simulink library "pmm"  (R2021b)
settings: Solver=VariableStepAuto  StartTime=0.0  StopTime=10.0  RelTol=1e-3
undefined symbols (not defined in the file or in its folder): APMM_CoolgFanActCurr_X_pct, APMM_EWP1Curr_X_c, APMM_EWP3Curr_X_c, APMM_LVBattChktime_X_enum, APMM_LVBattChrgtime_X_enum, APMM_LVChrgLv24V_X_mV, APMM_LVChrgLv_X_mV, ENUM_ANTITHEFT_ALARM, ENUM_ANTITHEFT_ARM, ENUM_ANTITHEFT_DISARM, ENUM_ANTITHEFT_WAIT, ENUM_CHRGPLUGSTA_NONE, ENUM_CRASHSTATE_NOCRASH, ENUM_DCDCFAULTSTA_ANYFAULTLV1, ENUM_DCDCFAULTSTA_ANYFAULTLV2, ENUM_DRIVETRAIN_AWD, ENUM_DRIVETRAIN_FWD, ENUM_DRIVETRAIN_RWD, ENUM_EBSBRKSW_PRESSED, ENUM_GEARACTUALPOSN_D, ENUM_GEARACTUALPOSN_N, ENUM_GEARACTUALPOSN_P, ENUM_GEARACTUALPOSN_R, ENUM_HVBATTREADYPRE_READY, ENUM_PDKEYRAWLULOCK_INLOCK, ENUM_PDKEYRAWLULOCK_INUNLOCK, ENUM_PDKEYRAWPS_INPS, ENUM_PDKEYSTA_LOCK, ENUM_PDKEYSTA_PS, ENUM_PDKEYSTA_UNAVALIABLE, ENUM_PDKEYSTA_UNLOCK, ENUM_POWERSTA_OFF, ENUM_POWERSTA_OFFA, ENUM_POWERSTA_OFFC, ENUM_POWERSTA_ON, ENUM_POWERSTA_READY, ENUM_POWERSTA_STANDBY, ENUM_PWRSTASW_PWRUP, ENUM_PWRSTASW_READY, FALSE, KPMM_AllDoorClosedHoldTime_s, KPMM_APSAllowThd_pct, KPMM_BattDownFailtime_s, KPMM_BattUpFailtime_s, KPMM_BattUpResetRty_cnt, KPMM_BattUpResetSW_flg, KPMM_BattUpResetTO_s, KPMM_BattUpRstDlyTO_s, KPMM_BrakeSWHoldTime_s, KPMM_ChrgPlugHoldTime_s, KPMM_DCDCDisableFailtime_s, KPMM_DCDCEnableFailtime_s, KPMM_DCDCVSET_V, KPMM_DCDCVSETLVChrg_V, KPMM_DoorSWHoldTime_s, KPMM_DriverSafetyChkFailtime_s, KPMM_DrivetrainSelect_enum_ovrdflg, KPMM_DrivetrainSelect_enum_ovrdval, KPMM_FDADC12VDetAccu_s, KPMM_FDADC12VDetAccuIntval_s ... (+60)
libraries: simulink x35, hcu_lib x13
(part 5 of 6)

== stateflow chart pmm/PMM/PMM/PMM_State_Machine ==
  state OFF
    en:
    VPMM_LVPwrSta_flg = FALSE;
    VPMM_PowerSta_enum = ENUM_POWERSTA_OFF;
    VPMM_PwrStaSW_enum = ENUM_PWRSTASW_OFF;
    VPMM_LVSilentChrgSta_enum = ENUM_SILENTCHRGSTA_NONE;
    VPMM_LVSilentChrgReq_flg = FALSE;
    VPMM_LVSilentChrgReqStd_flg = FALSE;
    VPMM_PreOFF_flg = TRUE;
    VPMM_PwrStaTOSta_enum = ENUM_PWRSTATOSTA_NORMAL;
    VPMM_PowerUpState_enum = ENUM_PUSTATE_INITIALIZE;
    VPMM_FirstLVCheckHoldTimer_s = 0;
    VPMM_24VFirstLVCheckHoldTimer_s = 0;
    VPMM_PMMAllowECUSleep_flg = FALSE;
    VPMM_SilentChrgFaultBypass_flg = FALSE;
    VPMM_FDADC12VDetAvg_mV = 0;
    VPMM_FDADC24VDetAvg_mV = 0;
    VPMM_SilentChkAllowSleep_flg = FALSE;
    ex:
    VPMM_PMMAllowECUSleep_flg = FALSE;
    VPMM_PMMAllowNMSleep_flg = FALSE;
    state LVBatt_Check_Wake_Hold [parallel]
      en:
      VPMM_LVBattChkWakeholdTimer_s = 0;
      VPMM_TimerAllowSleep_flg = FALSE;
      settings: executionOrder=1
      (default) -> (junction 3132)
      (junction 3132) -> (junction 3133) [order 1] : [VPMM_LVBattChkWakeholdTimer_s >= KPMM_LVBattChkWakehold_s]
      LVBatt_Check_Wake_Hold -> (junction 3132)
      (junction 3132) -> (junction 3134) [order 2] : {
          |  VPMM_LVBattChkWakeholdTimer_s += task_time_s;
          |  VPMM_TimerAllowSleep_flg = FALSE;
          | }
      (junction 3133) -> (junction 3135) : {VPMM_TimerAllowSleep_flg = TRUE;
          |  VPMM_LVBattChkWakeholdTimer_s = KPMM_LVBattChkWakehold_s;}
      (junction 3135) -> (junction 3134)
    state Silent_Charge_Judge [parallel]
      en:
      VPMM_SilentChkAllowSleep12V_flg = FALSE;
      settings: executionOrder=2
      state SilentChrgLv = SilentChrgLvCal(LVBatt_mV) [function]
      state LVBatStaChk
        en:
        VPMM_FDADC12VDetAccuTimer_s = 0;
        VPMM_OFFLVBattChkRechk_cnt = 0;
        VPMM_FDADC12VDetAccu_cnt = 0;
        VPMM_FDADC12VDetbuff_mV = 0;
        VPMM_FDADC12VDetAvgTMP_mV = 0;
        VPMM_OFFLVBattChkRechkDone_flg = FALSE;
        VPMM_LVBatStaChk_flg = 0;
        (default) -> (junction 3179)
        OFF.Silent_Charge_Judge.LVBatStaChk -> (junction 3179) [order 1]
        (junction 3179) -> (junction 3180) [order 1] : [VPMM_FirstLVCheckHoldTimer_s >= KPMM_FirstLVCheckHoldT_s]
        (junction 3180) -> (junction 3181) : {VPMM_FirstLVCheckHoldTimer_s = KPMM_FirstLVCheckHoldT_s;}
        (junction 3179) -> (junction 3195) [order 2] : {
            |  VPMM_FirstLVCheckHoldTimer_s += task_time_s;
            |  VPMM_OFFLVBattChkRechkDone_flg = FALSE;
            |  VPMM_SilentChkAllowSleep12V_flg = FALSE;
            |  }
        (junction 3181) -> (junction 3182) [order 1] : [VPMM_FDADC12VDetAccuTimer_s >= ...
            | (VPMM_FDADC12VDetAccu_cnt * KPMM_FDADC12VDetAccuIntval_s)]
        (junction 3181) -> (junction 3183) [order 2]
        (junction 3182) -> (junction 3184) : {VPMM_FDADC12VDetbuff_mV += VINP_LvBattVolt_mV;
            |  VPMM_FDADC12VDetAccu_cnt++;}
        (junction 3184) -> (junction 3183)
        (junction 3183) -> (junction 3185)
        (junction 3185) -> (junction 3186) [order 1] : [VPMM_FDADC12VDetAccuTimer_s >= KPMM_FDADC12VDetAccu_s]
        (junction 3185) -> (junction 3196) [order 2] : {VPMM_FDADC12VDetAccuTimer_s += task_time_s;}
        (junction 3186) -> (junction 3405)
        (junction 3405) -> (junction 3406) [order 1] : [VPMM_FDADC12VDetAccu_cnt <= 0]
        (junction 3405) -> (junction 3410) [order 2] : {VPMM_FDADC12VDetAvgTMP_mV = VPMM_FDADC12VDetbuff_mV / VPMM_FDADC12VDetAccu_cnt;}
        (junction 3406) -> (junction 3412) : {VPMM_FDADC12VDetAvgTMP_mV = VINP_LvBattVolt_mV;}
        (junction 3412) -> (junction 3410)
        (junction 3410) -> (junction 3187)
        (junction 3187) -> (junction 3188) [order 1] : [VPMM_FirstFDADC12VDetAvg_mV <= 0]
        (junction 3187) -> (junction 3189) [order 2]
        (junction 3188) -> (junction 3190) : {VPMM_FirstFDADC12VDetAvg_mV = VPMM_FDADC12VDetAvgTMP_mV;}
        (junction 3190) -> (junction 3189)
        (junction 3189) -> (junction 3191) : {VPMM_FDADC12VDetAvg_mV = VPMM_FDADC12VDetAvgTMP_mV;}
        (junction 3191) -> (junction 3192) [order 1] : [VPMM_FDADC12VDetAvgTMP_mV < KPMM_LVBattOFFSlpThd_mV]
        (junction 3191) -> (junction 3197) [order 2] : {
            |  VPMM_LVBatStaChk_flg = TRUE;
            | }
        (junction 3192) -> (junction 3193) : {VPMM_LVBatStaChk_flg = FALSE;}
        (junction 3193) -> (junction 3194) [order 1] : [VPMM_OFFLVBattChkRechk_cnt >= KPMM_OFFLVBattChkRetry_cnt ]
        (junction 3193) -> (junction 3198) [order 2] : {
            |  VPMM_OFFLVBattChkRechkDone_flg = FALSE;
            |  VPMM_OFFLVBattChkRechk_cnt++;
            |  VPMM_FDADC12VDetAccuTimer_s = 0;
            |  VPMM_FDADC12VDetAccu_cnt = 0;
            |  VPMM_FDADC12VDetbuff_mV = 0;
            |  VPMM_FDADC12VDetAvgTMP_mV = 0;}
        (junction 3194) -> (junction 3199) : {VPMM_OFFLVBattChkRechkDone_flg = TRUE;}
        (junction 3196) -> (junction 3195)
        (junction 3197) -> (junction 3196)
        (junction 3198) -> (junction 3197)
        (junction 3199) -> (junction 3198)
      state HoodOffStaChk [commented out]
        en:
        VPMM_HoodOffStaChk_flg = FALSE;
        (default) -> (junction 3255) [commented out] : {VPMM_HoodOffChkFailtimer_s = 0;}
        OFF.Silent_Charge_Judge.HoodOffStaChk -> (junction 3255) [commented out]
        (junction 3255) -> (junction 3256) [commented out] : [!VINP_HoodSW_flg]
        (junction 3256) -> (junction 3258) [commented out] : {VPMM_HoodOffStaChk_flg = TRUE;}
        (junction 3255) -> (junction 3257) [commented out] : {VPMM_HoodOffChkFailtimer_s += task_time_s;}
        (junction 3258) -> (junction 3257) [commented out]
        (junction 3257) -> (junction 3259) [commented out]
      state CANMsgValid
        en:
        VPMM_CANMsgValid_flg = FALSE;
        (default) -> (junction 3229) : {VPMM_CANValidChkFailtimer_s = 0;}
        OFF.Silent_Charge_Judge.CANMsgValid -> (junction 3229) [order 1]
        (junction 3229) -> (junction 3230) [order 1] : [VINP_CANMsgValidBMS3_flg && VINP_CANMsgValidBMS5_flg]
        (junction 3229) -> (junction 3231) [order 2] : {VPMM_CANValidChkFailtimer_s += task_time_s;}
        (junction 3230) -> (junction 3232) : {VPMM_CANMsgValid_flg = TRUE;}
        (junction 3232) -> (junction 3231)
        (junction 3231) -> (junction 3233)
      state HVBSOCOffStaChk
        en:
        VPMM_HVBSOCOffStaChk_flg = FALSE;
        (default) -> (junction 3242) : {VPMM_HVBSOCOffStaChkFailtimer_s = 0;}
        (junction 3242) -> (junction 3243) [order 1] : [VINP_HVBattSOC_pct > KPMM_HVBattSOCThd_pct]
        OFF.Silent_Charge_Judge.HVBSOCOffStaChk -> (junction 3242) [order 1]
        (junction 3242) -> (junction 3244) [order 2] : {VPMM_HVBSOCOffStaChkFailtimer_s += task_time_s;}
        (junction 3243) -> (junction 3245) : {VPMM_HVBSOCOffStaChk_flg = TRUE;}
        (junction 3245) -> (junction 3244)
        (junction 3244) -> (junction 3246)
      state Silent_Charge_Allow_Sleep
        en:
        VPMM_LVSilentChrgLv12V_enum = SilentChrgLvCal(VPMM_FDADC12VDetAvg_mV);
        VPMM_SilentChkAllowSleep12V_flg = TRUE;
        VPMM_LVSilentChrgReq12V_flg = FALSE;
        VPMM_PMMAllowNMSleep12V_flg = TRUE;
      state Silent_Charge_Need_Wake
        en:
        VPMM_LVSilentChrgLv12V_enum = SilentChrgLvCal(VPMM_FDADC12VDetAvg_mV);
        %VPMM_LVChrgReqCnt_cnt++;
        VPMM_SilentChkAllowSleep12V_flg = FALSE;
        VPMM_LVSilentChrgReq12V_flg = TRUE;
      (default) -> (junction 3144)
      (junction 3143) -> (junction 3144)
      (junction 3144) -> (junction 3145) [order 1] : [!KPMM_OFFStaByPassLVBatt_flg]
      (junction 3150) -> (junction 3143)
      (junction 3144) -> OFF.Silent_Charge_Judge.Silent_Charge_Allow_Sleep [order 2]
      (junction 3145) -> OFF.Silent_Charge_Judge.LVBatStaChk
      OFF.Silent_Charge_Judge.LVBatStaChk -> (junction 3146) [order 2] : [VPMM_LVBatStaChk_flg == TRUE]
      (junction 3146) -> (junction 3149)
      OFF.Silent_Charge_Judge.LVBatStaChk -> (junction 3438) [order 1] : [VPMM_LVBatStaChk_flg == FALSE &&...
          |  VPMM_OFFLVBattChkRechkDone_flg == TRUE]
      (junction 3149) -> (junction 3440)
      OFF.Silent_Charge_Judge.HoodOffStaChk -> ? [commented out] : [VPMM_HoodOffChkFailtimer_s >= KPMM_HoodOffChkFailtime_s]
          | {VPMM_LVSilentChrgSta_enum = ENUM_SILENTCHRGSTA_FAULT;}
      OFF.Silent_Charge_Judge.HoodOffStaChk -> ? [commented out] : [VPMM_HoodOffStaChk_flg]
      (junction 3438) -> (junction 3440) [commented out] : [VPMM_SilentChrgFaultBypass_flg]
      (junction 3438) -> OFF.Silent_Charge_Judge.CANMsgValid : {VPMM_PMMAllowNMSleep12V_flg = FALSE;}
      (junction 3440) -> (junction 3147)
      OFF.Silent_Charge_Judge.CANMsgValid -> (junction 3147) [order 2] : [VPMM_CANValidChkFailtimer_s >= KPMM_CANValidChkFailtime_s]
          | {VPMM_LVSilentChrgSta_enum = ENUM_SILENTCHRGSTA_FAULT;
          |  VPMM_SilentChrgFaultBypass_flg = TRUE;}
      (junction 3147) -> (junction 3148)
      OFF.Silent_Charge_Judge.CANMsgValid -> OFF.Silent_Charge_Judge.HVBSOCOffStaChk [order 1] : [VPMM_CANMsgValid_flg]
      OFF.Silent_Charge_Judge.HVBSOCOffStaChk -> (junction 3148) [order 2] : [VPMM_HVBSOCOffStaChkFailtimer_s >= KPMM_HVBSOCOffStaChkFailtime_s]
          | {VPMM_LVSilentChrgSta_enum = ENUM_SILENTCHRGSTA_FAULT;
          |  VPMM_SilentChrgFaultBypass_flg = TRUE;}
      (junction 3148) -> (junction 3355)
      OFF.Silent_Charge_Judge.HVBSOCOffStaChk -> (junction 3354) [order 1] : [VPMM_HVBSOCOffStaChk_flg]
      (junction 3354) -> (junction 3355) [order 2] : {VPMM_LVSilentChrgSta_enum = ENUM_SILENTCHRGSTA_FAULT;
          |  VPMM_SilentChrgFaultBypass_flg = TRUE;}
      (junction 3355) -> OFF.Silent_Charge_Judge.Silent_Charge_Allow_Sleep
      (junction 3354) -> OFF.Silent_Charge_Judge.Silent_Charge_Need_Wake [order 1] : [VPMM_PowerUpFault_enum == ENUM_PUFAULT_NOFAULT]
      OFF.Silent_Charge_Judge.Silent_Charge_Allow_Sleep -> (junction 3151)
      OFF.Silent_Charge_Judge.Silent_Charge_Need_Wake -> (junction 3152)
      (junction 3151) -> (junction 3150)
      (junction 3152) -> (junction 3151)
    state Silent_Charge_Judge24V [parallel]
      en:
      VPMM_SilentChkAllowSleep24V_flg = FALSE;
      settings: executionOrder=3
      state SilentChrgLv24V = SilentChrgLvCal24V(LVBatt24V_mV) [function]
      state LVBatStaChk
        en:
        VPMM_FDADC24VDetAccuTimer_s = 0;
        VPMM_24VOFFLVBattChkRechk_cnt = 0;
        VPMM_FDADC24VDetAccu_cnt = 0;
        VPMM_FDADC24VDetbuff_mV = 0;
        VPMM_FDADC24VDetAvgTMP_mV = 0;
        VPMM_24VOFFLVBattChkRechkDone_flg = FALSE;
        VPMM_24VLVBatStaChk_flg = 0;
        (default) -> (junction 3872)
        OFF.Silent_Charge_Judge24V.LVBatStaChk -> (junction 3872) [order 1]
        (junction 3872) -> (junction 3873) [order 1] : [VPMM_24VFirstLVCheckHoldTimer_s >= KPMM_FirstLVCheckHoldT_s]
        (junction 3872) -> (junction 3892) [order 2] : {
            |  VPMM_24VFirstLVCheckHoldTimer_s += task_time_s;
            |  VPMM_24VOFFLVBattChkRechkDone_flg = FALSE;
            |  VPMM_SilentChkAllowSleep24V_flg = FALSE;
            |  }
        (junction 3873) -> (junction 3874) : {VPMM_24VFirstLVCheckHoldTimer_s = KPMM_FirstLVCheckHoldT_s;}
        (junction 3874) -> (junction 3875) [order 1] : [VPMM_FDADC24VDetAccuTimer_s >= ...
            | (VPMM_FDADC24VDetAccu_cnt * KPMM_FDADC24VDetAccuIntval_s)]
        (junction 3874) -> (junction 3876) [order 2]
        (junction 3875) -> (junction 3877) : {VPMM_FDADC24VDetbuff_mV += VINP_LvBattVolt24V_mV;
            |  VPMM_FDADC24VDetAccu_cnt++;}
        (junction 3877) -> (junction 3876)
        (junction 3876) -> (junction 3878)
        (junction 3878) -> (junction 3879) [order 1] : [VPMM_FDADC24VDetAccuTimer_s >= KPMM_FDADC24VDetAccu_s]
        (junction 3878) -> (junction 3893) [order 2] : {VPMM_FDADC24VDetAccuTimer_s += task_time_s;}
        (junction 3879) -> (junction 3880)
        (junction 3880) -> (junction 3881) [order 1] : [VPMM_FDADC24VDetAccu_cnt <= 0]
        (junction 3880) -> (junction 3882) [order 2] : {VPMM_FDADC24VDetAvgTMP_mV = VPMM_FDADC24VDetbuff_mV / VPMM_FDADC24VDetAccu_cnt;}
        (junction 3881) -> (junction 3883) : {VPMM_FDADC24VDetAvgTMP_mV = VINP_LvBattVolt24V_mV;}
        (junction 3883) -> (junction 3882)
        (junction 3882) -> (junction 3884)
        (junction 3884) -> (junction 3885) [order 1] : [VPMM_FirstFDADC24VDetAvg_mV <= 0]
        (junction 3884) -> (junction 3886) [order 2]
        (junction 3885) -> (junction 3887) : {VPMM_FirstFDADC24VDetAvg_mV = VPMM_FDADC24VDetAvgTMP_mV;}
        (junction 3887) -> (junction 3886)
        (junction 3886) -> (junction 3888) : {VPMM_FDADC24VDetAvg_mV = VPMM_FDADC24VDetAvgTMP_mV;}
        (junction 3888) -> (junction 3889) [order 1] : [VPMM_FDADC24VDetAvgTMP_mV < KPMM_LVBattOFFSlpThd24V_mV]
        (junction 3888) -> (junction 3894) [order 2] : {
            |  VPMM_24VLVBatStaChk_flg = TRUE;
            | }
        (junction 3889) -> (junction 3890) : {VPMM_24VLVBatStaChk_flg = FALSE;}
        (junction 3890) -> (junction 3891) [order 1] : [VPMM_24VOFFLVBattChkRechk_cnt >= KPMM_OFFLVBattChkRetry_cnt ]
        (junction 3890) -> (junction 3895) [order 2] : {
            |  VPMM_24VOFFLVBattChkRechkDone_flg = FALSE;
            |  VPMM_24VOFFLVBattChkRechk_cnt++;
            |  VPMM_FDADC24VDetAccuTimer_s = 0;
            |  VPMM_FDADC24VDetAccu_cnt = 0;
            |  VPMM_FDADC24VDetbuff_mV = 0;
            |  VPMM_FDADC24VDetAvgTMP_mV = 0;}
        (junction 3891) -> (junction 3896) : {VPMM_24VOFFLVBattChkRechkDone_flg = TRUE;}
        (junction 3893) -> (junction 3892)
        (junction 3894) -> (junction 3893)
        (junction 3895) -> (junction 3894)
        (junction 3896) -> (junction 3895)
      state HoodOffStaChk [commented out]
        en:
        VPMM_HoodOffStaChk_flg = FALSE;
        (default) -> (junction 3931) [commented out] : {VPMM_HoodOffChkFailtimer_s = 0;}
        OFF.Silent_Charge_Judge24V.HoodOffStaChk -> (junction 3931) [commented out]
        (junction 3931) -> (junction 3932) [commented out] : [!VINP_HoodSW_flg]
        (junction 3932) -> (junction 3934) [commented out] : {VPMM_HoodOffStaChk_flg = TRUE;}
        (junction 3931) -> (junction 3933) [commented out] : {VPMM_HoodOffChkFailtimer_s += task_time_s;}
        (junction 3934) -> (junction 3933) [commented out]
        (junction 3933) -> (junction 3935) [commented out]
      state CANMsgValid
        en:
        VPMM_24VCANMsgValid_flg = FALSE;
        (default) -> (junction 3944) : {VPMM_24VCANValidChkFailtimer_s = 0;}
        OFF.Silent_Charge_Judge24V.CANMsgValid -> (junction 3944) [order 1]
        (junction 3944) -> (junction 3945) [order 1] : [VINP_CANMsgValidBMS3_flg && VINP_CANMsgValidDCDCStatus2_flg]
        (junction 3944) -> (junction 3946) [order 2] : {VPMM_24VCANValidChkFailtimer_s += task_time_s;}
        (junction 3945) -> (junction 3947) : {VPMM_24VCANMsgValid_flg = TRUE;}
        (junction 3947) -> (junction 3946)
        (junction 3946) -> (junction 3948)
      state HVBSOCOffStaChk
        en:
        VPMM_HVBSOCOffStaChk_flg = FALSE;
        (default) -> (junction 3957) : {VPMM_HVBSOCOffStaChkFailtimer_s = 0;}
        (junction 3957) -> (junction 3958) [order 1] : [VINP_HVBattSOC_pct > KPMM_HVBattSOCThd_pct]
        OFF.Silent_Charge_Judge24V.HVBSOCOffStaChk -> (junction 3957) [order 1]
        (junction 3957) -> (junction 3959) [order 2] : {VPMM_HVBSOCOffStaChkFailtimer_s += task_time_s;}
        (junction 3958) -> (junction 3960) : {VPMM_HVBSOCOffStaChk_flg = TRUE;}
        (junction 3960) -> (junction 3959)
        (junction 3959) -> (junction 3961)
      state Silent_Charge_Allow_Sleep
        en:
        VPMM_LVSilentChrgLv24V_enum = SilentChrgLvCal24V(VPMM_FDADC24VDetAvg_mV);
        VPMM_SilentChkAllowSleep24V_flg = TRUE;
        VPMM_LVSilentChrgReq24V_flg = FALSE;
        VPMM_PMMAllowNMSleep24V_flg = TRUE;
      state Silent_Charge_Need_Wake
        en:
        VPMM_LVSilentChrgLv24V_enum = SilentChrgLvCal24V(VPMM_FDADC24VDetAvg_mV);
        %VPMM_LVChrgReqCnt_cnt++;
        VPMM_SilentChkAllowSleep24V_flg = FALSE;
        VPMM_LVSilentChrgReq24V_flg = TRUE;
      (default) -> (junction 3827)
      (junction 3826) -> (junction 3827)
      (junction 3827) -> (junction 3828) [order 1] : [!KPMM_OFFStaByPassLVBatt_flg]
      (junction 3837) -> (junction 3826)
      (junction 3827) -> OFF.Silent_Charge_Judge24V.Silent_Charge_Allow_Sleep [order 2]
      (junction 3828) -> OFF.Silent_Charge_Judge24V.LVBatStaChk
      OFF.Silent_Charge_Judge24V.LVBatStaChk -> (junction 3829) [order 2] : [VPMM_24VLVBatStaChk_flg == TRUE]
      (junction 3829) -> (junction 3830)
      OFF.Silent_Charge_Judge24V.LVBatStaChk -> (junction 3832) [order 1] : [VPMM_24VLVBatStaChk_flg == FALSE &&...
          |  VPMM_24VOFFLVBattChkRechkDone_flg == TRUE]
      (junction 3830) -> (junction 3831)
      OFF.Silent_Charge_Judge24V.HoodOffStaChk -> ? [commented out] : [VPMM_HoodOffChkFailtimer_s >= KPMM_HoodOffChkFailtime_s]
          | {VPMM_LVSilentChrgSta_enum = ENUM_SILENTCHRGSTA_FAULT;}
      OFF.Silent_Charge_Judge24V.HoodOffStaChk -> ? [commented out] : [VPMM_HoodOffStaChk_flg]
      (junction 3832) -> (junction 3831) [commented out] : [VPMM_SilentChrgFaultBypass_flg]
      (junction 3831) -> (junction 3833)
      (junction 3832) -> OFF.Silent_Charge_Judge24V.CANMsgValid : {VPMM_PMMAllowNMSleep24V_flg = FALSE;}
      OFF.Silent_Charge_Judge24V.CANMsgValid -> (junction 3833) [order 2] : [VPMM_24VCANValidChkFailtimer_s >= KPMM_CANValidChkFailtime_s]
          | {VPMM_LVSilentChrgSta_enum = ENUM_SILENTCHRGSTA_FAULT;
          |  VPMM_SilentChrgFaultBypass_flg = TRUE;}
      (junction 3833) -> (junction 3834)
      OFF.Silent_Charge_Judge24V.CANMsgValid -> OFF.Silent_Charge_Judge24V.HVBSOCOffStaChk [order 1] : [VPMM_24VCANMsgValid_flg]
      OFF.Silent_Charge_Judge24V.HVBSOCOffStaChk -> (junction 3834) [order 2] : [VPMM_HVBSOCOffStaChkFailtimer_s >= KPMM_HVBSOCOffStaChkFailtime_s]
          | {VPMM_LVSilentChrgSta_enum = ENUM_SILENTCHRGSTA_FAULT;
          |  VPMM_SilentChrgFaultBypass_flg = TRUE;}
      (junction 3834) -> (junction 3835)
      OFF.Silent_Charge_Judge24V.HVBSOCOffStaChk -> (junction 3836) [order 1] : [VPMM_HVBSOCOffStaChk_flg]
      (junction 3836) -> (junction 3835) [order 2] : {VPMM_LVSilentChrgSta_enum = ENUM_SILENTCHRGSTA_FAULT;
          |  VPMM_SilentChrgFaultBypass_flg = TRUE;}
      (junction 3835) -> OFF.Silent_Charge_Judge24V.Silent_Charge_Allow_Sleep
      (junction 3836) -> OFF.Silent_Charge_Judge24V.Silent_Charge_Need_Wake [order 1] : [VPMM_PowerUpFault_enum == ENUM_PUFAULT_NOFAULT]
      OFF.Silent_Charge_Judge24V.Silent_Charge_Allow_Sleep -> (junction 3838)
      OFF.Silent_Charge_Judge24V.Silent_Charge_Need_Wake -> (junction 3839)
      (junction 3838) -> (junction 3837)
      (junction 3839) -> (junction 3838)
    state Data_Handler [parallel]
      settings: executionOrder=4
      state Lv = GetMaxLv(Lv12, Lv24) [function]
      (default) -> (junction 3988)
      Data_Handler -> (junction 3988)
      (junction 3988) -> (junction 3990) [order 1] : [VPMM_SilentChkAllowSleep12V_flg && VPMM_SilentChkAllowSleep24V_flg]
      (junction 3988) -> (junction 3994) [order 2] : {VPMM_SilentChkAllowSleep_flg = FALSE;}
      (junction 3990) -> (junction 3992) : {VPMM_SilentChkAllowSleep_flg = TRUE;}
      (junction 3992) -> (junction 3994)
      (junction 3994) -> (junction 4006)
      (junction 4006) -> (junction 4007) [order 1] : [VPMM_LVSilentChrgReq12V_flg || VPMM_LVSilentChrgReq24V_flg]
      (junction 4006) -> (junction 4009) [order 2] : {VPMM_LVSilentChrgReq_flg = FALSE;}
      (junction 4007) -> (junction 4011) : {VPMM_LVSilentChrgReq_flg = TRUE;}
      (junction 4011) -> (junction 4009)
      (junction 4009) -> (junction 4014) : {VPMM_LVSilentChrgLv_enum = GetMaxLv(VPMM_LVSilentChrgLv12V_enum,VPMM_LVSilentChrgLv24V_enum);}
    state PMM_Allow_ECU_Sleep_Judge [parallel]
      settings: executionOrder=5
      state LVBattChktimeOut = LVBattChkTimeCal(SilentChrgLv) [function]
      (default) -> (junction 3270)
      PMM_Allow_ECU_Sleep_Judge -> (junction 3270)
      (junction 3270) -> (junction 3271) [order 1] : [VPMM_TimerAllowSleep_flg &&...
          |  VPMM_SilentChkAllowSleep_flg]
      (junction 3271) -> (junction 3273) : {VPMM_PMMAllowECUSleep_flg = TRUE;
          |  VPMM_LVBattChktime_s = LVBattChkTimeCal(VPMM_LVSilentChrgLv_enum);}
      (junction 3270) -> (junction 3272) [order 2] : {VPMM_PMMAllowECUSleep_flg = FALSE;}
      (junction 3273) -> (junction 3272)
  state Stand_By
    en:
    VPMM_PwrStaSW_enum = ENUM_PWRSTASW_STANDBY;
    VPMM_PowerSta_enum = ENUM_POWERSTA_STANDBY;
    VPMM_PrePwrSta_enum = ENUM_POWERSTA_STANDBY;
    VPMM_PwrStaTOSta_enum = ENUM_PWRSTATOSTA_NORMAL;
    VPMM_LVPwrSta_flg = TRUE;
    VPMM_PwrStaStdTOtimer_s = 0;
    VPMM_LVBattChkOKStdTtimer_s = 0;
    ex:
    VPMM_PreOFF_flg = FALSE;
    VPMM_PwrStaTOSta_enum = ENUM_PWRSTATOSTA_NORMAL;
    (default) -> (junction 3360)
    Stand_By -> (junction 3360) [order 1]
    (junction 3360) -> (junction 3361) [order 1] : [VPMM_LVSilentChrgReq_flg]
    (junction 3360) -> (junction 3363) [order 2]
    (junction 3361) -> (junction 3362)
    (junction 3363) -> (junction 3364) [order 1] : [KPMM_SilentChrgReq_flg_ovrdflg]
    (junction 3363) -> (junction 3365) [order 2]
    (junction 3364) -> (junction 3369) : {VPMM_LVSilentChrgReqStd_flg = KPMM_SilentChrgReq_flg_ovrdval;}
    (junction 3365) -> (junction 3366) [order 1] : [(VINP_LVBattDet12V_V < KPMM_LVBattThd_V ||...
        |   VINP_LVBattDet24V_V < KPMM_LVBattThd24V_V) && ...
        |  VPMM_PowerUpState_enum != ENUM_PUSTATE_POWERUPFAIL]
    (junction 3365) -> (junction 3371) [order 2] : {VPMM_LVBattChkOKStdTtimer_s = 0;}
    (junction 3366) -> (junction 3367)
    (junction 3367) -> (junction 3368) [order 1] : [VPMM_LVBattChkOKStdTtimer_s >= KPMM_LVBattChkOKStdT_s]
    (junction 3368) -> (junction 3369) [order 1] : [VINP_HVBattSOC_pct > KPMM_HVBattSOCThd_pct && !VINP_HoodSW_flg]
        | {VPMM_LVSilentChrgReqStd_flg = TRUE;}
    (junction 3367) -> (junction 3370) [order 2] : {VPMM_LVBattChkOKStdTtimer_s += task_time_s;}
    (junction 3368) -> (junction 3372) [order 2] : {VPMM_LVSilentChrgSta_enum = ENUM_SILENTCHRGSTA_FAULT;}
    (junction 3369) -> (junction 3379) : {VPMM_LVSilentChrgSta_enum = ENUM_SILENTCHRGSTA_NONE;}
    (junction 3371) -> (junction 3372)
    (junction 3372) -> (junction 3373) [order 1] : [VINP_PwrReq_OTA_enum == ENUM_PWRREQOTA_REQPOWERSTDBY]
    (junction 3372) -> (junction 3375) [order 2]
    (junction 3373) -> (junction 3374)
    (junction 3375) -> (junction 3376) [order 1] : [VPMM_PwrStaStdTOtimer_s >= KPMM_PwrStaStdTO_s]
    (junction 3375) -> (junction 3377) [order 2] : {VPMM_PwrStaStdTOtimer_s += task_time_s;
        |  VPMM_PwrStaTOSta_enum = ENUM_PWRSTATOSTA_NORMAL;}
    (junction 3376) -> (junction 3378) : {VPMM_PwrStaTOSta_enum = ENUM_PWRSTATOSTA_TIMEOUT;
        |  VPMM_PwrStaStdTOtimer_s = 0;}
  state PowerDown
    en:
    VPMM_PwrStaSW_enum = ENUM_PWRSTASW_PWRDOWN;
    VPMM_PowerDownState_enum = ENUM_PDSTATE_INITIALIZE;
    VPMM_PowerDownFault_enum = ENUM_PDFAULT_NOFAULT;
    VPMM_MLvSafetyPDCompleted_flg = FALSE;
    VPMM_MCUPDCompleted_flg = FALSE;
    VPMM_DCDCPDCompleted_flg = FALSE;
    VPMM_BattPDCompleted_flg = FALSE;
    VPMM_MCUDischrgComplete_flg = FALSE;
    VPMM_OBCPDCompleted_flg = FALSE;
    VPMM_Sched_ChgTOSta_enum = ENUM_SCHEDCHGTO_NORMAL;
    VPMM_PCUPwrDowFaultSta_enum = ENUM_PCUPDSTA_NORMAL;
    ex:
    VPMM_LVSilentChrgReq_flg = FALSE;
    VPMM_LVSilentChrgReqStd_flg = FALSE;
    VPMM_LVSilentChrgReq12V_flg = FALSE;
    VPMM_LVSilentChrgReq24V_flg = FALSE;
    state MLvSafetyPDCheck
      en:
      VPMM_PowerDownState_enum = ENUM_PDSTATE_MLVSAFETYCHK;
      (default) -> (junction 272) : {
          | VPMM_TimeMLvSafetyPDChk_s = 0;
          | }
      MLvSafetyPDCheck -> (junction 272) [order 1]
      (junction 272) -> (junction 273) [order 1] : [VPMM_SafetyChkMLv_flg]
      (junction 272) -> (junction 274) [order 2]
      (junction 273) -> (junction 278) : {
          | VPMM_MLvSafetyPDCompleted_flg = TRUE;
          | }
      (junction 274) -> (junction 275) [order 1] : [VPMM_TimeMLvSafetyPDChk_s >= KPMM_MLvSafetyFailtime_s]
      (junction 274) -> (junction 276) [order 2] : {
          | VPMM_TimeMLvSafetyPDChk_s += task_time_s;
          | }
      (junction 275) -> (junction 277) : {
          | VPMM_PowerDownFault_enum = ENUM_PDFAULT_MLVSAFETYFAIL;
          | VPMM_MLvSafetyPDCompleted_flg = TRUE;
          | }
      (junction 277) -> (junction 276)
      (junction 278) -> (junction 277)
    state MCUDisable
      en:
      VPMM_PowerDownState_enum = ENUM_PDSTATE_MCUDISABLE;
      (default) -> (junction 290) : {
          | VPMM_TimeMCUDisable_s = 0;
          | }
      MCUDisable -> (junction 290) [order 1]
      (junction 290) -> (junction 292) : %{VPMM_MCUEnaReq_flg = FALSE;}
      (junction 292) -> (junction 293) [order 1] : [!VPMM_MCUEnable_flg]
      (junction 292) -> (junction 294) [order 2]
      (junction 293) -> (junction 298) : {
          | VPMM_MCUPDCompleted_flg = TRUE;
          | }
      (junction 294) -> (junction 295) [order 1] : [VPMM_TimeMCUDisable_s >= KPMM_MCUDisableFailtime_s]
      (junction 294) -> (junction 296) [order 2] : {
          | VPMM_TimeMCUDisable_s += task_time_s;
          | }
      (junction 295) -> (junction 297) : {
          | VPMM_PowerDownFault_enum = ENUM_PDFAULT_MCUDISABLE;
          | VPMM_MCUPDCompleted_flg = TRUE;
          | }
      (junction 297) -> (junction 296)
      (junction 298) -> (junction 297)
    state DCDCDisable
      en:
      VPMM_PowerDownState_enum = ENUM_PDSTATE_DCDCDISABLE;
      (default) -> (junction 315) : {
          | VPMM_TimeDCDCDisable_s = 0;
          | }
      DCDCDisable -> (junction 315) [order 1]
      (junction 315) -> (junction 316) : {
          | VPMM_DCDCEnaReq_flg = FALSE;
          | }
      (junction 316) -> (junction 317) [order 1] : [!VINP_DCDCEnabled_flg]
      (junction 316) -> (junction 318) [order 2]
      (junction 317) -> (junction 322) : {
          | VPMM_DCDCPDCompleted_flg = TRUE;
          | }
      (junction 318) -> (junction 319) [order 1] : [VPMM_TimeDCDCDisable_s >= KPMM_DCDCDisableFailtime_s]
      (junction 318) -> (junction 320) [order 2] : {
          | VPMM_TimeDCDCDisable_s += task_time_s;
          | }
      (junction 319) -> (junction 321) : {
          | VPMM_PowerDownFault_enum = ENUM_PDFAULT_DCDCDISABLE;
          | VPMM_DCDCPDCompleted_flg = TRUE;
          | }
      (junction 321) -> (junction 320)
      (junction 322) -> (junction 321)
    state PCUPwrDown1
      en:
      %VPMM_PowerDownState_enum = ENUM_PDSTATE_DCDCDISABLE;
      (default) -> (junction 3602) : {
          | VPMM_PCUDCDCPD1Completed_flg = FALSE;
          | VPMM_TimePCUDCDCDisable_s = 0;
          | }
      PCUPwrDown1 -> (junction 3602) [order 1]
      (junction 3602) -> (junction 3603) : {
          | VPMM_DCDCEnDem_enum = ENUM_DCDCENDEM_SHUTDOWN;
          | }
      (junction 3603) -> (junction 3604) [order 1] : [VINP_DCDCEnSta_enum == ENUM_DCDCENSTA_READY &&...
          |  VINP_EHPSEnSta_enum == ENUM_EHPSENSTA_READY &&...
          |  VINP_EACEnSta_enum == ENUM_EACENSTA_READY]
      (junction 3603) -> (junction 3605) [order 2]
      (junction 3604) -> (junction 3609) : {
          | VPMM_PCUDCDCPD1Completed_flg = TRUE;
          | }
      (junction 3605) -> (junction 3606) [order 1] : [VPMM_TimePCUDCDCDisable_s >= KPMM_PCUChkFailTime_s]
      (junction 3605) -> (junction 3607) [order 2] : {
          | VPMM_TimePCUDCDCDisable_s += task_time_s;
          | }
      (junction 3606) -> (junction 3608) : {
          | VPMM_PCUPwrDowFaultSta_enum = ENUM_PCUPDSTA_PCUDISABLEFAIL;
          | VPMM_PCUDCDCPD1Completed_flg = TRUE;
          | }
      (junction 3608) -> (junction 3607)
      (junction 3609) -> (junction 3608)
    state BattPackPowerdown
      en:
      VPMM_PowerDownState_enum = ENUM_PDSTATE_BATTPACK;
      (default) -> (junction 335) : {
          | VPMM_TimeBattPD_s = 0;
          | }
      BattPackPowerdown -> (junction 335) [order 1]
      (junction 335) -> (junction 337) : {
          | VPMM_HVBatCnctReq_flg = FALSE;
          | }
      (junction 337) -> (junction 336) [order 1] : [!VINP_HVBContactorSta_flg]
      (junction 336) -> (junction 342) : {
          | %VPMM_HVPwrSta_flg = FALSE;
          | VPMM_BattPDCompleted_flg = TRUE;
          | }
      (junction 337) -> (junction 338) [order 2]
      (junction 338) -> (junction 339) [order 1] : [VPMM_TimeBattPD_s >= KPMM_BattDownFailtime_s]
      (junction 338) -> (junction 340) [order 2] : {
          | VPMM_TimeBattPD_s += task_time_s;
          | }
      (junction 339) -> (junction 341) : {
          | VPMM_PowerDownFault_enum = ENUM_PDFAULT_BATTPDFAIL;
          | VPMM_BattPDCompleted_flg = TRUE;
          | }
      (junction 341) -> (junction 340)
      (junction 342) -> (junction 341)
    state PCUPwrDown2
      en:
      %VPMM_PowerDownState_enum = ENUM_PDSTATE_DCDCDISABLE;
      (default) -> (junction 3633) : {
          | VPMM_PCUDCDCPD2Completed_flg = FALSE;
          | VPMM_TimePCUDCDCDisable_s = 0;
          | }
      PCUPwrDown2 -> (junction 3633) [order 1]
      (junction 3633) -> (junction 3634) : {
          | VPMM_DCDCRlyDem_enum = ENUM_DCDCRLYDEM_DISABLE;
          | VPMM_EACRlyDem_enum = ENUM_EACRLYDEM_DISABLE;
          | VPMM_EHPSRlyDem_enum = ENUM_EHPSRLYDEM_DISABLE;
          | }
      (junction 3634) -> (junction 3635) [order 1] : [VINP_PDUDCDCRlySta_enum == ENUM_PDUDCDCRLYSTA_OPEN &&...
          |  VINP_PDUEACRlySta_enum == ENUM_PDUEACRLYSTA_OPEN &&...
          |  VINP_PDUEHPSRlySta_enum == ENUM_PDUEHPSRLYSTA_OPEN]
      (junction 3634) -> (junction 3636) [order 2]
      (junction 3635) -> (junction 3640) : {
          | VPMM_PCUDCDCPD2Completed_flg = TRUE;
          | }
      (junction 3636) -> (junction 3637) [order 1] : [VPMM_TimePCUDCDCDisable_s >= KPMM_PCUChkFailTime_s]
      (junction 3636) -> (junction 3638) [order 2] : {
          | VPMM_TimePCUDCDCDisable_s += task_time_s;
          | }
      (junction 3637) -> (junction 3639) : {
          | VPMM_PCUPwrDowFaultSta_enum = ENUM_PCUPDSTA_PCURELAYOPENFAIL;
          | VPMM_PCUDCDCPD2Completed_flg = TRUE;
          | }
      (junction 3639) -> (junction 3638)
      (junction 3640) -> (junction 3639)
    state MCUDischrg
      en:
      VPMM_PowerDownState_enum = ENUM_PDSTATE_MCUDISCHRG;
      (default) -> (junction 355) : {
          | VPMM_TimeMCUDisChrg_s = 0;
          | }
      MCUDischrg -> (junction 355) [order 1]
      (junction 355) -> (junction 356) : {
          | VPMM_ActiveDischargeReq_flg = TRUE;
          | }
      (junction 356) -> (junction 357) [order 1] : [VPMM_MCUDCBusMaxVolt_V <= KPMM_MCUDischrgVolt_V]
          | %Modify condition from"VPMM_MCUDischrgFinished_flg"
          | % to "VPMM_MCUDCBusMaxVolt_V <= KPMM_MCUDischrgVolt_V"
      (junction 356) -> (junction 358) [order 2]
      (junction 357) -> (junction 362) : {
          | VPMM_MCUDischrgComplete_flg = TRUE;
          | VPMM_ActiveDischargeReq_flg = FALSE;
          | }
      (junction 358) -> (junction 359) [order 1] : [VPMM_TimeMCUDisChrg_s >= KPMM_MCUDisChrgFailtime_s]
      (junction 358) -> (junction 360) [order 2] : {
          | VPMM_TimeMCUDisChrg_s += task_time_s;
          | }
      (junction 359) -> (junction 361) : {
          | VPMM_PowerDownFault_enum = ENUM_PDFAULT_MCUDISCHRG;
          | VPMM_MCUDischrgComplete_flg = TRUE;
          | VPMM_ActiveDischargeReq_flg = FALSE;
          | }
      (junction 361) -> (junction 360)
      (junction 362) -> (junction 361)
    state OBCDisable
      en:
      VPMM_PowerDownState_enum = ENUM_PDSTATE_OBCDISABLE;
      (default) -> (junction 375) : {
          | VPMM_TimeOBCDisable_s = 0;
          | }
      OBCDisable -> (junction 375) [order 1]
      (junction 375) -> (junction 377) : {
          | VPMM_HVSysReadyToCharge_enum = ENUM_CHRGREADY_DISCHARGE;
          | }
      (junction 377) -> (junction 376) [order 1] : [!VINP_OBCEnabled_flg]
      (junction 376) -> (junction 382) : {
          | VPMM_OBCPDCompleted_flg = TRUE;
          | }
      (junction 377) -> (junction 378) [order 2]
      (junction 378) -> (junction 379) [order 1] : [VPMM_TimeOBCDisable_s >= KPMM_OBCDisableFailtime_s]
      (junction 378) -> (junction 380) [order 2] : {
          | VPMM_TimeOBCDisable_s += task_time_s;
          | }
      (junction 379) -> (junction 381) : {
          | VPMM_PowerDownFault_enum = ENUM_PDFAULT_OBCDISABLE;
          | VPMM_OBCPDCompleted_flg = TRUE;
          | }
      (junction 381) -> (junction 380)
      (junction 382) -> (junction 381)
    state PowerdownComplte
      en:
      VPMM_PowerDownState_enum = ENUM_PDSTATE_COMPLETE;
      VPMM_HVPwrSta_flg = FALSE;
      %VPMM_PowerDownCompleted_flg = TRUE;
      %Check if need VPMM_PowerDownCompleted_flg
    (default) -> (junction 255)
    (junction 255) -> (junction 256) [order 1] : [!VPMM_SafetyChkHLv_flg]
    (junction 255) -> MLvSafetyPDCheck [order 2]
    (junction 256) -> (junction 258) : {
        | %VPMM_MCUEnaReq_flg = FALSE;
        | }
    MLvSafetyPDCheck -> MCUDisable [order 1] : [VPMM_MLvSafetyPDCompleted_flg]
    MCUDisable -> DCDCDisable [order 1] : [VPMM_MCUPDCompleted_flg]
    DCDCDisable -> (junction 257) [order 1] : [VPMM_DCDCPDCompleted_flg]
    (junction 258) -> (junction 257)
    (junction 257) -> PCUPwrDown1
    PCUPwrDown1 -> BattPackPowerdown [order 1] : [VPMM_PCUDCDCPD1Completed_flg]
    BattPackPowerdown -> PCUPwrDown2 [order 1] : [VPMM_BattPDCompleted_flg]
    PCUPwrDown2 -> MCUDischrg [order 1] : [VPMM_PCUDCDCPD2Completed_flg]
    MCUDischrg -> OBCDisable [order 1] : [VPMM_MCUDischrgComplete_flg]
    OBCDisable -> PowerdownComplte [order 1] : [VPMM_OBCPDCompleted_flg]
  state PowerUp
    en:
    VPMM_PwrStaSW_enum = ENUM_PWRSTASW_PWRUP;
    VPMM_PowerUpState_enum = ENUM_PUSTATE_INITIALIZE;
    VPMM_PowerUpFault_enum = ENUM_PUFAULT_NOFAULT;
    VPMM_SafetyChkCompleted_flg = FALSE;
    VPMM_DrvSafetyChkCompleted_flg = FALSE;
    VPMM_HVSysChkCompleted_flg = FALSE;
    VPMM_BattPUCompleted_flg = FALSE;
    VPMM_DCDCPUCompleted_flg = FALSE;
    VPMM_DCDCSetVCompleted_flg = FALSE;
    %VPMM_PowerUpComplete_flg = FALSE;
    %VPMM_PowerUpFail_flg = FALSE;
    VPMM_PCUPwrUpFaultSta_enum = ENUM_PCUPUSTA_NORMAL;
    note: ENUM_PWRSTASW_PWRDOWN
    note: ENUM_PWRSTASW_PWRDOWN
    state SafetyCheck
      en:
      VPMM_PowerUpState_enum = ENUM_PUSTATE_SAFETYCHK;
      (default) -> (junction 422) : {
          | VPMM_TimeSafetyChk_s = 0;
          | }
      SafetyCheck -> (junction 422) [order 1]
      (junction 422) -> (junction 423) [order 1] : [(VPMM_SafetyChkMLv_flg && ...
          |   VPMM_SafetyChkHLv_flg)]
      (junction 422) -> (junction 424) [order 2] : {
          | VPMM_TimeSafetyChk_s += task_time_s;
          | }
      (junction 423) -> (junction 425) : {
          | VPMM_SafetyChkCompleted_flg = TRUE;
          | }
      (junction 425) -> (junction 424)
    state DriverSafetyCheck
      en:
      VPMM_PowerUpState_enum = ENUM_PUSTATE_DRVSAFETYCHK;
      (default) -> (junction 433) : {
          | VPMM_TimeDrvSafetyChk_s = 0;
          | }
      DriverSafetyCheck -> (junction 433) [order 1]
      (junction 433) -> (junction 434) [order 1] : [VTQD_GearActualPosn_enum == ENUM_GEARACTUALPOSN_P || ...
          |  VTQD_GearActualPosn_enum == ENUM_GEARACTUALPOSN_N]
      (junction 433) -> (junction 435) [order 2] : {
          | VPMM_TimeDrvSafetyChk_s += task_time_s;
          | }
      (junction 434) -> (junction 436) : {
          | VPMM_DrvSafetyChkCompleted_flg = TRUE;
          | }
      (junction 436) -> (junction 435)
    state HVSysCheck
      en:
      VPMM_PowerUpState_enum = ENUM_PUSTATE_HVSYSCHK;
      (default) -> (junction 444) : {
          | VPMM_TimeHVSysChk_s = 0;
          | }
      HVSysCheck -> (junction 444) [order 1]
      (junction 444) -> (junction 445) [order 1] : [VPMM_PreChrgChk_flg]
      (junction 444) -> (junction 446) [order 2] : {
          | VPMM_TimeHVSysChk_s += task_time_s;
          | }
      (junction 445) -> (junction 447) : {
          | VPMM_HVSysChkCompleted_flg = TRUE;
          | }
      (junction 447) -> (junction 446)
    state BattPackPowerup
      en:
      VPMM_PowerUpState_enum = ENUM_PUSTATE_BATTPACK;
      (default) -> (junction 455) : {
          | VPMM_TimeBattPU_s = 0;
          | }
      BattPackPowerup -> (junction 455) [order 1]
      (junction 455) -> (junction 456) : {
          | VPMM_HVBatCnctReq_flg = TRUE;
          | }
      (junction 456) -> (junction 457) [order 1] : [VINP_HVBContactorSta_flg && VINP_BMSREADY_flg ]
      (junction 456) -> (junction 458) [order 2] : {
          | VPMM_TimeBattPU_s += task_time_s;
          | }
      (junction 457) -> (junction 459) : {
          | VPMM_BattPUCompleted_flg = TRUE;
          | }
      (junction 459) -> (junction 458)
    state HardwareResetProcess
      en:
      VPMM_BattUpResetTO_s = 0;
      VPMM_BattUpRstDlyTO_s = 0;
      VPMM_HWResetSta_enum = 0;
      VPMM_HVBatCnctReq_flg = FALSE;
      VPMM_HardwareRst_flg = FALSE;
      (default) -> (junction 3075)
      HardwareResetProcess -> (junction 3075) [order 1] : [VPMM_BattUpReset_flg]
          | {VPMM_BattUpReset_flg = FALSE;}
      (junction 3075) -> (junction 3081) : {VPMM_HWResetSta_enum = 1;
          |  VPMM_CtrlDrPwrStbA2_flg = TRUE;
          |  VPMM_CtrlFrPwrStbA1P_flg = TRUE;
          |  VPMM_CtrlFrRC1_flg = TRUE;
          |  VPMM_CtrlFrBMSCCUCIR_flg = TRUE;
          |  VPMM_CtrlFrEDUINVERTER_flg = TRUE;}
      (junction 3081) -> (junction 3087) [order 1] : [VPMM_BattUpResetTO_s >= KPMM_BattUpResetTO_s]
      (junction 3081) -> (junction 3085) [order 2] : {VPMM_BattUpResetTO_s += task_time_s;
          |  VPMM_BattUpReset_flg = TRUE;}
      (junction 3087) -> (junction 3089) : {VPMM_HWResetSta_enum = 2;
          |  VPMM_CtrlDrPwrStbA2_flg = FALSE;
          |  VPMM_CtrlFrPwrStbA1P_flg = FALSE;
          |  VPMM_CtrlFrRC1_flg = FALSE;
          |  VPMM_CtrlFrBMSCCUCIR_flg = FALSE;
          |  VPMM_CtrlFrEDUINVERTER_flg = FALSE;}
      HardwareResetProcess -> (junction 3089) [order 2]
      (junction 3089) -> (junction 3091) [order 1] : [VPMM_BattUpRstDlyTO_s >= KPMM_BattUpRstDlyTO_s]
      (junction 3089) -> (junction 3093) [order 2] : {VPMM_BattUpRstDlyTO_s += task_time_s;}
      (junction 3091) -> (junction 3095) : {VPMM_HardwareRst_flg = TRUE;}
      (junction 3093) -> (junction 3095)
    state DCDCEnable
      en:
      VPMM_PowerUpState_enum = ENUM_PUSTATE_DCDCENABLE;
      (default) -> (junction 468) : {
          | VPMM_TimeDCDCEnable_s = 0;
          | }
      DCDCEnable -> (junction 468) [order 1]
      (junction 468) -> (junction 469) : {
          | VPMM_DCDCEnaReq_flg = TRUE;
          | }
      (junction 469) -> (junction 470) [order 1] : [VINP_DCDCEnabled_flg]
      (junction 470) -> (junction 472) : {
          | VPMM_DCDCPUCompleted_flg = TRUE;
          | }
      (junction 469) -> (junction 471) [order 2] : {
          | VPMM_TimeDCDCEnable_s += task_time_s;
          | }
      (junction 472) -> (junction 471)
    state PCU_PwrUp_Delay
      (default) -> (junction 3449) : {
          | VPMM_TimePCUDelay_s = 0;
          | VPMM_PCUPwrUpDelayDone_flg = FALSE;
          | }
      (junction 3449) -> (junction 3450) [order 1] : [VPMM_TimePCUDelay_s >= KPMM_PCUPwrUpDelayTime_s]
      PCU_PwrUp_Delay -> (junction 3449) [order 1]
      (junction 3449) -> (junction 3451) [order 2] : {
          | VPMM_TimePCUDelay_s += task_time_s;
          | }
      (junction 3450) -> (junction 3452) : {
          | VPMM_PCUPwrUpDelayDone_flg = TRUE;
          | }
      (junction 3452) -> (junction 3451)
    state PCU_DCDC_Relay
      en:
      %VPMM_PowerUpState_enum = ENUM_PUSTATE_DCDCENABLE;
      (default) -> (junction 3461) : {VPMM_PDUDCDCRlyDone_flg = FALSE;
          |  VPMM_TimePDUDCDCRlyEnable_s = 0;}
      PCU_DCDC_Relay -> (junction 3461) [order 1]
      (junction 3461) -> (junction 3501) [order 1] : [KPMM_PCUDCDCRlyEnByPassSW_flg]
      (junction 3461) -> (junction 3462) [order 2] : {VPMM_DCDCRlyDem_enum = ENUM_DCDCRLYDEM_ENABLE;}
      (junction 3501) -> (junction 3463)
      (junction 3462) -> (junction 3463) [order 1] : [VINP_PDUDCDCRlySta_enum == ENUM_PDUDCDCRLYSTA_CLOSE]
      (junction 3462) -> (junction 3464) [order 2] : {
          | VPMM_TimePDUDCDCRlyEnable_s += task_time_s;
          | }
      (junction 3463) -> (junction 3465) : {
          | VPMM_PDUDCDCRlyDone_flg = TRUE;
          | }
      (junction 3465) -> (junction 3464)
    state PCU_EAC_Relay
      en:
      %VPMM_PowerUpState_enum = ENUM_PUSTATE_DCDCENABLE;
      (default) -> (junction 3507) : {VPMM_PDUEACRlyDone_flg = FALSE;
          |  VPMM_TimePDUEACRlyEnable_s = 0;}
      PCU_EAC_Relay -> (junction 3507) [order 1]
      (junction 3507) -> (junction 3508) [order 1] : [KPMM_PCUEACRlyEnByPassSW_flg]
      (junction 3507) -> (junction 3509) [order 2] : {VPMM_EACRlyDem_enum = ENUM_EACRLYDEM_ENABLE;}
      (junction 3508) -> (junction 3510)
      (junction 3509) -> (junction 3510) [order 1] : [VINP_PDUEACRlySta_enum == ENUM_PDUEACRLYSTA_CLOSE]
      (junction 3509) -> (junction 3511) [order 2] : {
          | VPMM_TimePDUEACRlyEnable_s += task_time_s;
          | }
      (junction 3510) -> (junction 3512) : {
          | VPMM_PDUEACRlyDone_flg = TRUE;
          | }
      (junction 3512) -> (junction 3511)
    state PCU_EHPS_Relay
      en:
      %VPMM_PowerUpState_enum = ENUM_PUSTATE_DCDCENABLE;
      (default) -> (junction 3539) : {VPMM_PDUEHPSRlyDone_flg = FALSE;
          |  VPMM_TimePDUEHPSRlyEnable_s = 0;}
      PCU_EHPS_Relay -> (junction 3539) [order 1]
      (junction 3539) -> (junction 3540) [order 1] : [KPMM_PCUEHPSRlyEnByPassSW_flg]
      (junction 3539) -> (junction 3541) [order 2] : {VPMM_EHPSRlyDem_enum = ENUM_EHPSRLYDEM_ENABLE;}
      (junction 3540) -> (junction 3542)
      (junction 3541) -> (junction 3542) [order 1] : [VINP_PDUEHPSRlySta_enum == ENUM_PDUEHPSRLYSTA_CLOSE]
      (junction 3541) -> (junction 3543) [order 2] : {
          | VPMM_TimePDUEHPSRlyEnable_s += task_time_s;
          | }
      (junction 3542) -> (junction 3544) : {
          | VPMM_PDUEHPSRlyDone_flg = TRUE;
          | }
      (junction 3544) -> (junction 3543)
    state PCU_DCDC_Enable
      en:
      %VPMM_PowerUpState_enum = ENUM_PUSTATE_DCDCENABLE;
      (default) -> (junction 3556) : {VPMM_PDUDCDCEnableDone_flg = FALSE;
          |  VPMM_TimePDUDCDCEnable_s = 0;}
      PCU_DCDC_Enable -> (junction 3556) [order 1]
      (junction 3556) -> (junction 3557) [order 1] : [KPMM_PCUDCDCRlyEnByPassSW_flg]
      (junction 3557) -> (junction 3559)
      (junction 3556) -> (junction 3558) [order 2] : {VPMM_DCDCEnDem_enum = ENUM_DCDCENDEM_START;}
      (junction 3558) -> (junction 3559) [order 1] : [VINP_DCDCEnSta_enum == ENUM_DCDCENSTA_RUN]
      (junction 3558) -> (junction 3560) [order 2] : {
          | VPMM_TimePDUDCDCEnable_s += task_time_s;
          | }
      (junction 3559) -> (junction 3561) : {
          | VPMM_PDUDCDCEnableDone_flg = TRUE;
          | }
      (junction 3561) -> (junction 3560)
    state PowerUpComplete
      en:
      VPMM_PowerUpState_enum = ENUM_PUSTATE_COMPLETED;
      VPMM_HVPwrSta_flg = TRUE;
      VPMM_LVSilentChrgSta_enum = ENUM_SILENTCHRGSTA_NONE;
      %VPMM_PowerUpComplete_flg = TRUE;
      %Check if need PowerUpComplete_flg
    state Timeout
      en:
      VPMM_PowerUpState_enum = ENUM_PUSTATE_POWERUPFAIL;
      VPMM_HVPwrSta_flg = FALSE;
      %VPMM_PowerUpFail_flg = TRUE;
      %Check if need VPMM_PowerUpFail_flg
    (default) -> SafetyCheck
    SafetyCheck -> (junction 396) [order 2] : [VPMM_TimeSafetyChk_s >= KPMM_SafetyChkFailtime_s]
    (junction 396) -> Timeout : {VPMM_PowerUpFault_enum = ENUM_PUFAULT_SAFETYCHKFAIL;}
    SafetyCheck -> DriverSafetyCheck [order 1] : [VPMM_SafetyChkCompleted_flg]
    DriverSafetyCheck -> (junction 397) [order 2] : [VPMM_TimeDrvSafetyChk_s >= KPMM_DriverSafetyChkFailtime_s]
    (junction 397) -> Timeout : {VPMM_PowerUpFault_enum = ENUM_PUFAULT_DRVSAFETYCHKFAIL;}
    DriverSafetyCheck -> HVSysCheck [order 1] : [VPMM_DrvSafetyChkCompleted_flg]
    HVSysCheck -> (junction 398) [order 2] : [VPMM_TimeHVSysChk_s >= KPMM_PrechrgChkFailtime_s]
    (junction 398) -> Timeout : {VPMM_PowerUpFault_enum = ENUM_PUFAULT_PRECHRGCHKFAIL;}
    HVSysCheck -> BattPackPowerup [order 1] : [VPMM_HVSysChkCompleted_flg]
    HardwareResetProcess -> BattPackPowerup [order 1] : [VPMM_HardwareRst_flg]
    BattPackPowerup -> (junction 3118) [order 2] : [(VINP_BMSWarn6_flg && !KPMM_BattUpResetSW_flg) || ...
        |  VPMM_TimeBattPU_s >= KPMM_BattUpFailtime_s]
    (junction 3118) -> (junction 3126) [order 1] : [VINP_BMSWarn6_flg && !KPMM_BattUpResetSW_flg]
        | {VPMM_BattUpResetRty_cnt += 1;}
    (junction 3126) -> HardwareResetProcess [order 2]
    (junction 3118) -> (junction 3120) [order 2]
    (junction 3126) -> (junction 3127) [order 1] : [VPMM_BattUpResetRty_cnt >= KPMM_BattUpResetRty_cnt]
    BattPackPowerup -> DCDCEnable [order 1] : [VPMM_BattPUCompleted_flg]
    (junction 3127) -> (junction 3120)
    (junction 3120) -> Timeout : {VPMM_PowerUpFault_enum = ENUM_PUFAULT_BATTUPFAIL;}
    DCDCEnable -> (junction 400) [order 2] : [VPMM_TimeDCDCEnable_s >= KPMM_DCDCEnableFailtime_s]
    (junction 400) -> Timeout : {VPMM_PowerUpFault_enum = ENUM_PUFAULT_DCDCENABLEFAIL;}
    DCDCEnable -> PCU_PwrUp_Delay [order 1] : [VPMM_DCDCPUCompleted_flg]
        | {VPMM_DCDCVoltSetpointPU_V = KPMM_DCDCVSET_V;}
    PCU_PwrUp_Delay -> PCU_DCDC_Relay [order 1] : [VPMM_PCUPwrUpDelayDone_flg]
    PCU_DCDC_Relay -> (junction 3497) [order 2] : [VPMM_TimePDUDCDCRlyEnable_s >= KPMM_PCUChkFailTime_s]
    (junction 3497) -> Timeout : {VPMM_PCUPwrUpFaultSta_enum = ENUM_PCUPUSTA_DCDCRELAYFAIL;}
    PCU_DCDC_Relay -> PCU_EAC_Relay [order 1] : [VPMM_PDUDCDCRlyDone_flg]
    PCU_EAC_Relay -> (junction 3535) [order 2] : [VPMM_TimePDUEACRlyEnable_s >= KPMM_PCUChkFailTime_s]
    (junction 3535) -> Timeout : {VPMM_PCUPwrUpFaultSta_enum = ENUM_PCUPUSTA_EACRELAYFAIL;}
    PCU_EAC_Relay -> PCU_EHPS_Relay [order 1] : [VPMM_PDUEACRlyDone_flg]
    PCU_EHPS_Relay -> (junction 3573) [order 2] : [VPMM_TimePDUEHPSRlyEnable_s >= KPMM_PCUChkFailTime_s]
    (junction 3573) -> Timeout : {VPMM_PCUPwrUpFaultSta_enum = ENUM_PCUPUSTA_EHPSRELAYFAIL;}
    PCU_EHPS_Relay -> PCU_DCDC_Enable [order 1] : [VPMM_PDUEHPSRlyDone_flg]
    PCU_DCDC_Enable -> (junction 3578) [order 2] : [VPMM_TimePDUDCDCEnable_s >= KPMM_PCUChkFailTime_s]
    (junction 3578) -> Timeout : {VPMM_PCUPwrUpFaultSta_enum = ENUM_PCUPUSTA_24VDCDCENABLEFAIL;}
    PCU_DCDC_Enable -> PowerUpComplete [order 1] : [VPMM_PDUDCDCEnableDone_flg]
  state ON
    en:
    VPMM_PowerSta_enum = ENUM_POWERSTA_ON;
    VPMM_PrePwrSta_enum = ENUM_POWERSTA_ON;
    %VPMM_MCUEnaReq_flg = FALSE;
    VPMM_PwrStaTOSta_enum = ENUM_PWRSTATOSTA_NORMAL;
    VPMM_OBCPreChgChkFailtimer_s = 0;
    VPMM_PwrStaONTimer_s = 0;
    VPMM_PwrStaONTOPop_s = 0;
    VPMM_PwrStaONTOPopT_s = 0;
    VPMM_IVIPwrStaONTOPopT_s = 0;
    VPMM_ContinueUseHold_flg = FALSE;
    (default) -> (junction 7)
    ON -> (junction 7) [order 1]
    (junction 7) -> (junction 9) [order 1] : [VINP_OBCReady4Pre_flg]
        | {VPMM_OBCPreChgChkFailtimer_s = 0;}
    (junction 9) -> (junction 19) [order 1] : [VINP_OBCPluginSta_flg]
    (junction 7) -> (junction 11) [order 2]
    (junction 9) -> (junction 21) [order 2]
    (junction 19) -> (junction 26) : {VPMM_HVSysReadyToCharge_enum = ENUM_CHRGREADY_CHARGE;}
    (junction 11) -> (junction 21) [order 1] : [VPMM_OBCPreChgChkFailtimer_s >= KPMM_OBCPreChgChkFailtime_s]
        | {VPMM_HVChrgPreActionErrSta_enum = ENUM_CHGPREACTERRSTA_OBCPRE;}
    (junction 11) -> (junction 15) [order 2] : {VPMM_OBCPreChgChkFailtimer_s += task_time_s;}
    (junction 21) -> (junction 24) : {VPMM_HVSysReadyToCharge_enum = ENUM_CHRGREADY_DISCHARGE;}
    (junction 24) -> (junction 26)
    (junction 26) -> (junction 32) [order 1] : [VINP_ExtChrgSta_enum == ENUM_EXTCHRGSTS_CHARGING]
    (junction 26) -> (junction 2865) [order 2] : {VPMM_PwrStaSW_enum = ENUM_PWRSTASW_ON;}
    (junction 32) -> (junction 34) : {VPMM_PwrStaSW_enum = ENUM_PWRSTASW_ONHVCHRG;}
    (junction 2865) -> (junction 2866) [order 1] : [VINP_SeatSW_flg || ...
        |  VPMM_PwrStaConstraint_enum == ENUM_PWRCONSTRAINT_PWRSTAON || ...
        |  VPMM_PwrStaConstraint_enum == ENUM_PWRCONSTRAINT_ONFORTIME]
    (junction 2865) -> (junction 36) [order 2]
    (junction 2866) -> (junction 2870) : {VPMM_PwrStaONTimer_s = 0;
        |  VPMM_PwrStaONTOPop_s = 0;
        |  VPMM_IVIPwrStaONTOPopT_s = 0;}
    (junction 36) -> (junction 2873) [order 1] : [VPMM_PwrStaONTimer_s >= KPMM_PwrStaONTO_s - KPMM_PwrStaONTOPop_s]
    (junction 36) -> (junction 2009) [order 2] : {VPMM_PwrStaONTimer_s += task_time_s;
        |  VPMM_PwrStaTOSta_enum = ENUM_PWRSTATOSTA_NORMAL;
        |  VPMM_PwrStaONTOPop_s = 0;
        |  VPMM_PwrStaONTOPopReq_flg = FALSE;}
    (junction 2873) -> (junction 2875) : {VPMM_PwrStaONTOPop_s += task_time_s;
        |  VPMM_PwrStaONTOPopReq_flg = TRUE;
        |  VPMM_PwrStaONTOPopT_s = KPMM_PwrStaONTOPop_s - VPMM_PwrStaONTOPop_s;
        |  VPMM_IVIPwrStaONTOPopT_s = VPMM_PwrStaONTOPopT_s;
        |  VPMM_PwrStaONTimer_s += task_time_s;}
    (junction 2009) -> (junction 2875)
    (junction 2875) -> (junction 2877) [order 1] : [VPMM_ContinueUseHold_flg]
    (junction 2875) -> (junction 2879) [order 2]
    (junction 2877) -> (junction 2881)
    (junction 2879) -> (junction 2881) [order 1] : [VPMM_DetectPWCONTINUE_flg]
    (junction 2879) -> (junction 2886) [order 2] : {VPMM_ContinueUseHold_flg = FALSE;}
    (junction 2881) -> (junction 2884) : {VPMM_ContinueUseHold_flg = TRUE;
        |  VPMM_PwrStaONTimer_s = 0;
        |  VPMM_PwrStaONTOPop_s = 0;
        |  VPMM_IVIPwrStaONTOPopT_s = 0;}
    (junction 2886) -> (junction 2884) [order 2]
    (junction 2886) -> (junction 2007) [order 1] : [VPMM_PwrStaONTimer_s >= KPMM_PwrStaONTO_s]
        | {VPMM_PwrStaTOSta_enum = ENUM_PWRSTATOSTA_TIMEOUT;}
    (junction 2884) -> (junction 2889) : {VPMM_PwrStaTOSta_enum = ENUM_PWRSTATOSTA_NORMAL;}
  state OFF_A
    en:
    VPMM_PwrStaSW_enum = ENUM_PWRSTASW_OFFA;
    VPMM_PowerSta_enum = ENUM_POWERSTA_OFFA;
    VPMM_IVIPwrOffMemory_flg = VINP_IVIPwroffreq_flg;
    ex:
    VPMM_IVIPwrOffMemory_flg = FALSE;
  state OFF_C
    en:
    VPMM_PowerSta_enum = ENUM_POWERSTA_OFFC;
    VPMM_LVSilentChrgSta_enum = ENUM_SILENTCHRGSTA_NONE;
    VPMM_PrePwrSta_enum = ENUM_POWERSTA_OFFC;
    VPMM_PwrStaTOSta_enum = ENUM_PWRSTATOSTA_NORMAL;
    VPMM_Sched_ChgTOSta_enum = ENUM_SCHEDCHGTO_NORMAL;
    VPMM_LVBattChrgtime_s = LVBattChrgTimeCal(VPMM_LVSilentChrgLv_enum);
    VPMM_OFFCChkHVSOCLoop_flg = FALSE;
    VPMM_OBCPreChgChkFailtimer_s = 0;
    VPMM_LVBattChrgTimeCnt_s = 0;
    VPMM_PwrStaOFFCTimer_s = 0;
    VPMM_SchedChgTOTimer_s = 0;
    VPMM_LVChrgHoldTtimer_s = 0;
    VPMM_SilentChrgReqTimer_s = 0;
    state LVBattChrgTime= LVBattChrgTimeCal(SilentChrgLv) [function]
    state EWP1Curr = EWP1CurrCal(FDEWP1Cmd) [function]
    state EWP3Curr= EWP3CurrCal(FDEWP3Cmd) [function]
    state CoolgFanActCurr= CoolgFanActCurrCal(CoolgFanActDuty) [function]
    (default) -> (junction 1703)
    OFF_C -> (junction 1703) [order 2]
    (junction 1703) -> (junction 1704) [order 1] : [VINP_OBCReady4Pre_flg]
        | {VPMM_OBCPreChgChkFailtimer_s = 0;}
    (junction 1704) -> (junction 1705) [order 1] : [VINP_OBCPluginSta_flg]
    (junction 1703) -> (junction 1706) [order 2]
    (junction 1704) -> (junction 1707) [order 2]
    (junction 1705) -> (junction 1708) : {VPMM_HVSysReadyToCharge_enum = ENUM_CHRGREADY_CHARGE;}
    (junction 1706) -> (junction 1707) [order 1] : [VPMM_OBCPreChgChkFailtimer_s >= KPMM_OBCPreChgChkFailtime_s]
        | {VPMM_HVChrgPreActionErrSta_enum = ENUM_CHGPREACTERRSTA_OBCPRE;}
    (junction 1706) -> (junction 1710) [order 2] : {VPMM_OBCPreChgChkFailtimer_s +=task_time_s;}
    (junction 1707) -> (junction 1711) : {VPMM_HVSysReadyToCharge_enum = ENUM_CHRGREADY_DISCHARGE;}
    (junction 1708) -> (junction 1709) [order 1] : [VINP_ChrgPlugSta_enum != ENUM_CHRGPLUGSTA_NONE && ...
        |  (VINP_ExtChrgSta_enum == ENUM_EXTCHRGSTS_CHARGING || ...
        |   VINP_ExtChrgSta_enum == ENUM_EXTCHRGSTS_NOACTION)]
    (junction 1711) -> (junction 1708)
    (junction 1708) -> (junction 1712) [order 2]
    (junction 1709) -> (junction 1718) : {VPMM_PwrStaSW_enum = ENUM_PWRSTASW_OFFCHVCHRG;}
    (junction 1712) -> (junction 1713) [order 1] : [VPMM_LVSilentChrgReq_flg || ...
        |  VPMM_LVSilentChrgReqStd_flg]
    (junction 1712) -> (junction 2902) [order 2]
    (junction 1713) -> (junction 1715) : {VPMM_OFFCHVBattSOCTimer_s = 0;
        |  VPMM_SilentChrgReqTimer_s = 0;}
    (junction 2902) -> (junction 2906) [order 1] : [VPMM_SilentChrgReqTimer_s >= KPMM_SilentChrgReqTO_s]
    (junction 2902) -> (junction 2904) [order 2] : {VPMM_SilentChrgReqTimer_s += task_time_s;}
    (junction 2906) -> (junction 1714) : {VPMM_LVSilentChrgSta_enum = ENUM_SILENTCHRGSTA_FAULT;
        |  VPMM_LVSilentChrgReq_flg = FALSE;
        |  VPMM_LVSilentChrgReqStd_flg = FALSE;
        |  VPMM_SilentChrgReqTimer_s = 0;}
    OFF_C -> (junction 1715) [order 1] : [VPMM_OFFCChkHVSOCLoop_flg]
    (junction 1715) -> (junction 1716) [order 1] : [VINP_HVBattSOC_pct > KPMM_HVBattSOCThd_pct]
        | {VPMM_OFFCChkHVSOCLoop_flg = FALSE;}
    (junction 1716) -> (junction 2080) [order 1] : [!VINP_HoodSW_flg]
        | {VPMM_PwrStaSW_enum = ENUM_PWRSTASW_OFFCLVCHRG;}
    (junction 1718) -> (junction 2080) [order 1] : [VPMM_LVSilentChrgReq_flg || ...
        |  VPMM_LVSilentChrgReqStd_flg]
    (junction 1715) -> (junction 1719) [order 2]
    (junction 1716) -> (junction 1720) [order 2]
    (junction 2080) -> (junction 2825) : {VPMM_LVSilentChrgSta_enum = ENUM_SILENTCHRGSTA_CHARGING;}
    (junction 1718) -> (junction 1729) [order 2]
    (junction 1719) -> (junction 1720) [order 1] : [VPMM_OFFCHVBattSOCTimer_s >= KPMM_HVBSOCOFFCStaChkFailtime_s]
    (junction 1729) -> (junction 1987) [order 1] : [VINP_ExtChrgSta_enum == ENUM_EXTCHRGSTS_NOACTION]
    (junction 1987) -> (junction 2159) [order 1] : [VINP_SchedChgbutt_flg]
    (junction 1719) -> (junction 1724) [order 2] : {VPMM_OFFCHVBattSOCTimer_s += task_time_s;
        |  VPMM_OFFCChkHVSOCLoop_flg = TRUE;}
    (junction 1720) -> (junction 1725) : {VPMM_OFFCChkHVSOCLoop_flg = FALSE;
        |  VPMM_LVSilentChrgSta_enum = ENUM_SILENTCHRGSTA_FAULT;
        |  VPMM_LVSilentChrgReq_flg = FALSE;
        |  VPMM_LVSilentChrgReqStd_flg = FALSE;}
    (junction 1729) -> (junction 1991) [order 2]
    (junction 1987) -> (junction 1994) [order 2]
    (junction 2159) -> (junction 2166)
    (junction 2825) -> (junction 2826) [order 1] : [KPMM_LVChrgCurrMthd_flg]
        | {VPMM_EWP1Curr_A = EWP1CurrCal(VINP_FDEWP1Cmd_enum);
        |  VPMM_EWP3Curr_A = EWP3CurrCal(VINP_FDEWP3Cmd_enum);
        |  VPMM_CoolgFanActCurr_A = CoolgFanActCurrCal(VINP_CoolgFanActDuty_pct);
        |  VPMM_LVChrgCurrThd_A = VPMM_EWP1Curr_A + ...
        |  VPMM_EWP3Curr_A + ...
        |  VPMM_CoolgFanActCurr_A + ...
        |  KPMM_SysBaseCurr_A;}
    (junction 2826) -> (junction 2830) [order 1] : [VINP_DCDCAuxCur_A <= VPMM_LVChrgCurrThd_A]
    (junction 2830) -> (junction 2834) [order 1] : [VPMM_LVChrgHoldTtimer_s >= KPMM_LVChrgHoldT_s]
    (junction 2825) -> (junction 2828) [order 2]
    (junction 2826) -> (junction 1721) [order 2]
    (junction 2830) -> (junction 2832) [order 2] : {VPMM_LVChrgHoldTtimer_s += task_time_s;}
    (junction 2834) -> (junction 1722)
    (junction 1994) -> (junction 1996) [order 1] : [VPMM_PwrStaOFFCTimer_s >= KPMM_PwrStaOFFCTO_s]
    (junction 2166) -> (junction 2168) [order 1] : [VPMM_SchedChgTOTimer_s >= KPMM_Sched_ChgTO_s]
    (junction 1994) -> (junction 1993) [order 2] : {VPMM_PwrStaOFFCTimer_s += task_time_s;
        |  VPMM_PwrStaTOSta_enum = ENUM_PWRSTATOSTA_NORMAL;}
    (junction 1996) -> (junction 1995) : {VPMM_PwrStaTOSta_enum = ENUM_PWRSTATOSTA_TIMEOUT;
        |  VPMM_LVSilentChrgReq_flg = FALSE;
        |  VPMM_LVSilentChrgReqStd_flg = FALSE;}
    (junction 2166) -> (junction 2169) [order 2] : {VPMM_SchedChgTOTimer_s += task_time_s;
        |  VPMM_Sched_ChgTOSta_enum = ENUM_SCHEDCHGTO_NORMAL;}
    (junction 2168) -> (junction 2167) : {VPMM_Sched_ChgTOSta_enum = ENUM_SCHEDCHGTO_TIMEOUT;
        |  VPMM_LVSilentChrgReq_flg = FALSE;
        |  VPMM_LVSilentChrgReqStd_flg = FALSE;}
    (junction 2828) -> (junction 1721)
    (junction 1721) -> (junction 1722) [order 1] : [VPMM_LVBattChrgTimeCnt_s >= VPMM_LVBattChrgtime_s]
    (junction 1722) -> (junction 1723) [order 1] : [VINP_ExtChrgSta_enum == ENUM_EXTCHRGSTS_CHARGING]
    (junction 1721) -> (junction 1726) [order 2] : {VPMM_LVBattChrgTimeCnt_s += task_time_s;}
    (junction 1722) -> (junction 1727) [order 2] : {VPMM_LVSilentChrgSta_enum = ENUM_SILENTCHRGSTA_COMPLETE;
        |  VPMM_LVSilentChrgReq_flg = FALSE;
        |  VPMM_LVSilentChrgReqStd_flg = FALSE;}
    (junction 1723) -> (junction 1728)
  state Ready
    en:
    VPMM_PwrStaSW_enum = ENUM_PWRSTASW_READY;
    VPMM_PowerSta_enum = ENUM_POWERSTA_READY;
  (default) -> OFF : {VPMM_LVSilentChrgLv_enum = ENUM_SILENTCHRGLV_LV3;
      |  VPMM_FirstEnterOFF_flg = TRUE;
      |  VPMM_PMMAllowNMSleep_flg = TRUE;}
  (junction 1175) -> OFF : [VPMM_PowerDownState_enum == ENUM_PDSTATE_COMPLETE && ...
      |  VPMM_SafetyChkHLv_flg && ...
      |  VPMM_SafetyChkMLv_flg]
  PowerDown -> (junction 1175) [order 2]
  OFF -> Stand_By : [VPMM_OFFPBRisingEdge_flg || ...
      |  VPMM_PwrUpReq_enum == ENUM_PWRUPREQ_SYSREQPU || ...
      |  VINP_PwrReq_OTA_enum == ENUM_PWRREQOTA_REQPOWERSTDBY]
  Stand_By -> OFF [order 2] : [
      |  (VPMM_STBPBRisingEdge_flg || ...
      |   VPMM_PwrStaTOSta_enum == ENUM_PWRSTATOSTA_TIMEOUT || ...
      |   VPMM_DetectIVIPwroffreq_flg) && ...
      |  VPMM_PwrUpReq_enum != ENUM_PWRUPREQ_SYSREQPU && ...
      |  VINP_PwrReq_OTA_enum != ENUM_PWRREQOTA_REQPOWERSTDBY
      |  %&& !VPMM_BrkPedalPressed_flg
      | ]
  Stand_By -> (junction 1174) [order 1] : [VPMM_PwrUpReq_enum == ENUM_PWRUPREQ_USERREQPU || ...
      | VPMM_PwrUpReq_enum == ENUM_PWRUPREQ_SYSREQPU]
  (junction 1176) -> Stand_By : [VPMM_PowerDownState_enum == ENUM_PDSTATE_COMPLETE  && ...
      | (VPMM_PowerUpState_enum == ENUM_PUSTATE_POWERUPFAIL || ...
      | !VPMM_SafetyChkHLv_flg || ...
      | !VPMM_SafetyChkMLv_flg)]
  (junction 1174) -> PowerUp
  PowerDown -> (junction 1176) [order 1]
  PowerUp -> PowerDown [order 1] : [!VPMM_SafetyChkHLv_flg || ...
      |  !VPMM_SafetyChkMLv_flg]
      | {VPMM_PowerUpFault_enum = ENUM_PUFAULT_SAFETYCHKFAIL;}
  PowerUp -> PowerDown [order 2] : [VPMM_PowerUpState_enum == ENUM_PUSTATE_POWERUPFAIL || VPMM_PwrUpPBPress_flg]
      | %add20240729
  PowerUp -> (junction 1177) [order 4] : [VPMM_PowerUpState_enum == ENUM_PUSTATE_COMPLETED && ...
      |  VPMM_PwrStaSelect_enum == ENUM_PWRSTASELECT_GOOFFC]
  (junction 1177) -> OFF_C
  PowerUp -> (junction 1180) [order 3] : [VPMM_PowerUpState_enum == ENUM_PUSTATE_COMPLETED && ...
      |  VPMM_PwrStaSelect_enum == ENUM_PWRSTASELECT_GOON]
  (junction 1183) -> PowerDown
  (junction 1180) -> ON
  (junction 1179) -> (junction 1183)
  PowerUp -> (junction 1982) [order 5] : [
      |  VPMM_PowerUpState_enum == ENUM_PUSTATE_COMPLETED
      |  %&& VPMM_PwrStaSelect_enum == ENUM_PWRSTASELECT_GOOFFA
      | ]
  OFF_A -> PowerDown [order 3] : [VPMM_PwrDownReq_enum == ENUM_PWRDOWNREQ_USERREQPD || ...
      |  VPMM_PwrDownReq_enum == ENUM_PWRDOWNREQ_SYSREQPD || ...
      |  (!VPMM_SafetyChkHLv_flg || ...
      |   !VPMM_SafetyChkMLv_flg)]
  (junction 1982) -> (junction 1984)
  (junction 1984) -> OFF_A
  (junction 1131) -> (junction 1457)
  (junction 1457) -> (junction 1179)
  OFF_C -> (junction 1131) [order 1] : [!VPMM_SafetyChkHLv_flg || ...
      |  !VPMM_SafetyChkMLv_flg]
  (junction 1182) -> (junction 1457)
  ON -> (junction 1179) [order 1] : [!VPMM_SafetyChkHLv_flg || ...
      |  !VPMM_SafetyChkMLv_flg]
  ON -> OFF_C [order 4] : [((VPMM_ONPBRisingEdge_flg &&...
      |     VINP_FDDoorOpen_enum == ENUM_FDDOORSTA_OPEN &&...
      |     !VINP_SeatSW_flg) || VINP_IVIPwroffreq_flg)&&...
      |  VINP_ChrgPlugSta_enum != ENUM_CHRGPLUGSTA_NONE && ...
      |  (VPMM_PwrStaConstraint_enum != ENUM_PWRCONSTRAINT_PWRSTAON && ...
      |   VPMM_PwrStaConstraint_enum != ENUM_PWRCONSTRAINT_ONFORTIME)]
      | %add20240711
  OFF_A -> ON [order 1] : [VPMM_OFFAPBRisingEdge_flg || VINP_IVITriggerreq_flg || ...
      |  VPMM_BrkPedalRisingEdge_flg || VPMM_SeatSWRisingEdge_flg || ...
      |  ((VPMM_PwrStaConstraint_enum == ENUM_PWRCONSTRAINT_PWRSTAON || ...
      |    VPMM_PwrStaConstraint_enum == ENUM_PWRCONSTRAINT_ONFORTIME) && ...
      |   VPMM_PwrDownReq_enum != ENUM_PWRDOWNREQ_SYSREQPD)]
  OFF_C -> ON [order 2] : [VPMM_OFFCPBRisingEdge_flg || VINP_IVITriggerreq_flg || ...
      |  VPMM_BrkPedalRisingEdge_flg || VPMM_SeatSWRisingEdge_flg || ...
      |  VPMM_PwrStaConstraint_enum == ENUM_PWRCONSTRAINT_PWRSTAON || ...
      |  VPMM_PwrStaConstraint_enum == ENUM_PWRCONSTRAINT_ONFORTIME]
  ON -> OFF_A [order 3] : [(((VPMM_ONPBRisingEdge_flg &&...
      |     VINP_FDDoorOpen_enum == ENUM_FDDOORSTA_OPEN &&...
      |     !VINP_SeatSW_flg) ||...
      |     (VINP_IVIPwroffreq_flg || VPMM_READYPBMemory_flg)) &&...
      |    VINP_ChrgPlugSta_enum == ENUM_CHRGPLUGSTA_NONE &&...
      |    (VPMM_PwrStaConstraint_enum != ENUM_PWRCONSTRAINT_PWRSTAON && ...
      |     VPMM_PwrStaConstraint_enum != ENUM_PWRCONSTRAINT_ONFORTIME)) || ...
      |   VPMM_PwrDownReq_enum == ENUM_PWRDOWNREQ_SYSREQPD]
      | %add20240711
  OFF_C -> (junction 1115) [order 3] : [(VPMM_LVSilentChrgSta_enum == ENUM_SILENTCHRGSTA_COMPLETE ||...
      |   VPMM_LVSilentChrgSta_enum == ENUM_SILENTCHRGSTA_FAULT ||...
      |   VINP_ExtChrgSta_enum == ENUM_EXTCHRGSTS_COMPLETE ||...
      |   VINP_ExtChrgSta_enum == ENUM_EXTCHRGSTS_FAULT || ...
      |   VPMM_ChrgPlugFallingEdge_flg || ...
      |   VPMM_PwrStaTOSta_enum == ENUM_PWRSTATOSTA_TIMEOUT || ...
      |   VPMM_Sched_ChgTOSta_enum == ENUM_SCHEDCHGTO_TIMEOUT) && ...
      |   !VPMM_LVSilentChrgReq_flg && ...
      |   !VPMM_LVSilentChrgReqStd_flg]
  (junction 1117) -> OFF_C
  OFF_A -> (junction 1119) [order 2] : [VINP_ChrgPlugSta_enum != ENUM_CHRGPLUGSTA_NONE && ...
      |  VINP_ExtChrgSta_enum != ENUM_EXTCHRGSTS_COMPLETE && ...
      |  VINP_ExtChrgSta_enum != ENUM_EXTCHRGSTS_FAULT && ...
      |  VPMM_PwrStaTOSta_enum != ENUM_PWRSTATOSTA_TIMEOUT && ...
      |  VPMM_Sched_ChgTOSta_enum != ENUM_SCHEDCHGTO_TIMEOUT && ...
      |  VPMM_LVSilentChrgSta_enum != ENUM_SILENTCHRGSTA_COMPLETE && ...
      |  VPMM_LVSilentChrgSta_enum != ENUM_SILENTCHRGSTA_FAULT || ...
      |  (VINP_ChrgPlugSta_enum == ENUM_CHRGPLUGSTA_AC && ...
      |   VINP_ExtChrgSta_enum != ENUM_EXTCHRGSTS_COMPLETE && ...
      |   VINP_ExtChrgSta_enum != ENUM_EXTCHRGSTS_FAULT && ...
      |   VPMM_DetectSchedChg_flg)]
  (junction 1120) -> OFF_A
  ON -> Ready [order 2] : [
      |  VACC_EACPreSelfChkSta_flg &&...
      |  VINP_ChrgPlugSta_enum == ENUM_CHRGPLUGSTA_NONE && ...
      |  VPMM_MCUReady_flg && ...
      |  VINP_AllowMovThd_OTA_enum == ENUM_ALLOWMOV_ALLOWREADY && ...
      |  VDHP_ActAPSPosn_pct < KPMM_APSAllowThd_pct && ...
      |  VINP_V2LSta_enum == ENUM_V2LSTA_NOPLUG && ...
      |  VINP_PwrReq_OTA_enum != ENUM_PWRREQOTA_REQPOWERON &&...
      |  (VPMM_BrkPedalRisingEdge_flg &&...
      |   ((VPMM_PDKeySta_enum == ENUM_PDKEYSTA_PS) || VPMM_ONPBSta_flg))
      | ]
  Ready -> ON [order 1] : [
      |  ((VTQD_GearActualPosn_enum == ENUM_GEARACTUALPOSN_P || ...
      |    VTQD_EnterPGearFail_flg) && ...
      |   (VPMM_UserLeaveTChk_flg || VINP_IVIPwroffreq_flg || VINP_HVBattSOC_pct <= 0 || VINP_PwrReq_OTA_enum == ENUM_PWRREQOTA_REQPOWERON ||...
      |   (VINP_FDDoorOpen_enum == ENUM_FDDOORSTA_OPEN &&  !VINP_SeatSW_flg && VPMM_READYPBRisingEdge_flg))) || ...
      | ((VINP_ChrgPlugSta_enum != ENUM_CHRGPLUGSTA_NONE || ...
      |     VINP_V2LSta_enum != ENUM_V2LSTA_NOPLUG || ...
      |     (VINP_OFFACMODE_enum != ENUM_OFFACMODE_OFF && ...
      |      VINP_OFFACMODE_enum != ENUM_OFFACMODE_INVALID && ...
      |     VINP_HVBattSOC_pct < KPMM_HVSOCWarnThd_pct)) && ...
      |     VINP_VehSpeed_kph < KPMM_PluginVehSpdThd_kph)
      |  ]
  Ready -> (junction 1182) [order 2] : [!VPMM_SafetyChkHLv_flg || ...
      |  !VPMM_SafetyChkMLv_flg]
  (junction 1119) -> (junction 1117)
  (junction 1115) -> (junction 1120)
  data: LVBatt_mV function_input; SilentChrgLv function_output; LVBatt24V_mV function_input; SilentChrgLv24V function_output; Lv12 function_input; Lv24 function_input; Lv function_output; SilentChrgLv function_input; LVBattChktimeOut function_output; SilentChrgLv function_input; LVBattChrgTime function_output; FDEWP1Cmd function_input; EWP1Curr function_output; FDEWP3Cmd function_input; EWP3Curr function_output; CoolgFanActDuty function_input; CoolgFanActCurr function_output; VPMM_PowerUpState_enum output; VPMM_PowerDownState_enum output; VPMM_PowerUpFault_enum output; VPMM_PowerDownFault_enum output; VPMM_ActiveDischargeReq_flg output; VPMM_DCDCEnaReq_flg output; VPMM_DCDCVoltSetpointPU_V output single; VPMM_HVBatCnctReq_flg output; VPMM_HVSysReadyToCharge_enum output; VPMM_PowerSta_enum output; VPMM_LVPwrSta_flg output; VPMM_HVPwrSta_flg output; VPMM_PwrStaSW_enum output; task_time_s input; KPMM_BattUpFailtime_s input; KPMM_DCDCEnableFailtime_s input; KPMM_BattDownFailtime_s input; KPMM_MCUDisableFailtime_s input; KPMM_DCDCDisableFailtime_s input; KPMM_OBCDisableFailtime_s input; VINP_BMSREADY_flg input; VINP_ExtChrgSta_enum input; VPMM_DetectAntitheftUnlock_flg input; VINP_ChrgPlugSta_enum input; VINP_HVBContactorSta_flg input; VPMM_DetectDoorOpened_flg input; VPMM_MCUEnable_flg input; VPMM_PreChrgChk_flg input; VPMM_AllDoorClosed_flg input; VPMM_BrkPedalPressed_flg input; VPMM_MCUReady_flg input; VPMM_BrkPedalRisingEdge_flg input; VINP_OBCReady4Pre_flg input; VINP_OBCEnabled_flg input; VPMM_SafetyChkHLv_flg input; VPMM_SafetyChkMLv_flg input; VINP_LVBattDet12V_V input; VINP_IVITriggerreq_flg input; VPMM_PDKeySta_enum input; VINP_SeatSW_flg input; VINP_HVBattSOC_pct input; VTQD_GearActualPosn_enum input; KPMM_LVBattThd_V input; KPMM_HVBattSOCThd_pct input; KPMM_HVBSOCOffStaChkFailtime_s input; KPMM_HVBSOCOFFCStaChkFailtime_s input; KPMM_OBCPreChgChkFailtime_s input; KPMM_SafetyChkFailtime_s input; KPMM_DriverSafetyChkFailtime_s input; KPMM_PrechrgChkFailtime_s input; KPMM_MLvSafetyFailtime_s input; KPMM_MCUDisChrgFailtime_s input; KPMM_DCDCVSET_V input; VINP_DCDCEnabled_flg input; VINP_IVIPwroffreq_flg input; VPMM_AllDoorCloseRisingEdge_flg input; VTQD_EnterPGearFail_flg input; KPMM_SilentChrgReq_flg_ovrdflg input; KPMM_SilentChrgReq_flg_ovrdval input; VPMM_BattPDCompleted_flg local boolean; VPMM_BattPUCompleted_flg local boolean; VPMM_DCDCPDCompleted_flg local boolean; VPMM_DCDCPUCompleted_flg local boolean; VPMM_DrvSafetyChkCompleted_flg local boolean; VPMM_HVBSOCOffStaChkFailtimer_s local single; VPMM_HVBSOCOffStaChk_flg local boolean; VPMM_HVSysChkCompleted_flg local boolean; VPMM_LVChrgReqCnt_cnt local double; VPMM_MCUDischrgComplete_flg local boolean; VPMM_MCUPDCompleted_flg local boolean; VPMM_MLvSafetyPDCompleted_flg local boolean; VPMM_OBCPDCompleted_flg local boolean; VPMM_OBCPreChgChkFailtimer_s local single; VPMM_OFFCChkHVSOCLoop_flg local boolean; VPMM_OFFCHVBattSOCTimer_s local single; VPMM_SafetyChkCompleted_flg local boolean; VPMM_TimeBattPD_s local single; VPMM_TimeBattPU_s local single; VPMM_TimeDCDCDisable_s local single; VPMM_TimeDCDCEnable_s local single; VPMM_TimeDrvSafetyChk_s local single; VPMM_TimeHVSysChk_s local single; VPMM_TimeMCUDisChrg_s local single; VPMM_TimeMCUDisable_s local single; VPMM_TimeMLvSafetyPDChk_s local single; VPMM_TimeOBCDisable_s local single; VPMM_TimeSafetyChk_s local single; ENUM_CHGPREACTERRSTA_OBCPRE parameter; ENUM_CHRGPLUGSTA_NONE parameter; ENUM_CHRGREADY_CHARGE parameter; ENUM_CHRGREADY_DISCHARGE parameter; ENUM_EXTCHRGSTS_CHARGING parameter; ENUM_EXTCHRGSTS_COMPLETE parameter; ENUM_EXTCHRGSTS_FAULT parameter; ENUM_EXTCHRGSTS_NOACTION parameter; ENUM_GEARACTUALPOSN_N parameter; ENUM_GEARACTUALPOSN_P parameter; ENUM_PDFAULT_BATTPDFAIL parameter; ENUM_PDFAULT_DCDCDISABLE parameter; ENUM_PDFAULT_MCUDISABLE parameter; ENUM_PDFAULT_MCUDISCHRG parameter; ENUM_PDFAULT_MLVSAFETYFAIL parameter; ENUM_PDFAULT_NOFAULT parameter; ENUM_PDFAULT_OBCDISABLE parameter; ENUM_PDKEYSTA_PS parameter; ENUM_PDKEYSTA_UNLOCK parameter; ENUM_PDSTATE_BATTPACK parameter; ENUM_PDSTATE_COMPLETE parameter; ENUM_PDSTATE_DCDCDISABLE parameter; ENUM_PDSTATE_INITIALIZE parameter; ENUM_PDSTATE_MCUDISABLE parameter; ENUM_PDSTATE_MCUDISCHRG parameter; ENUM_PDSTATE_MLVSAFETYCHK parameter; ENUM_PDSTATE_OBCDISABLE parameter; ENUM_POWERSTA_OFF parameter; ENUM_POWERSTA_OFFA parameter; ENUM_POWERSTA_OFFC parameter; ENUM_POWERSTA_ON parameter; ENUM_POWERSTA_READY parameter; ENUM_POWERSTA_STANDBY parameter; ENUM_PUFAULT_BATTUPFAIL parameter; ENUM_PUFAULT_DCDCENABLEFAIL parameter; ENUM_PUFAULT_DRVSAFETYCHKFAIL parameter; ENUM_PUFAULT_NOFAULT parameter; ENUM_PUFAULT_PRECHRGCHKFAIL parameter; ENUM_PUFAULT_SAFETYCHKFAIL parameter; ENUM_PUSTATE_BATTPACK parameter; ENUM_PUSTATE_COMPLETED parameter; ENUM_PUSTATE_DCDCENABLE parameter; ENUM_PUSTATE_DRVSAFETYCHK parameter; ENUM_PUSTATE_HVSYSCHK parameter; ENUM_PUSTATE_INITIALIZE parameter; ENUM_PUSTATE_POWERUPFAIL parameter; ENUM_PUSTATE_SAFETYCHK parameter; ENUM_PWRSTASW_OFF parameter; ENUM_PWRSTASW_OFFA parameter; ENUM_PWRSTASW_OFFCHVCHRG parameter; ENUM_PWRSTASW_OFFCLVCHRG parameter; ENUM_PWRSTASW_ON parameter; ENUM_PWRSTASW_ONHVCHRG parameter; ENUM_PWRSTASW_PWRDOWN parameter; ENUM_PWRSTASW_PWRUP parameter; ENUM_PWRSTASW_READY parameter; ENUM_PWRSTASW_STANDBY parameter; ENUM_SILENTCHRGSTA_CHARGING parameter; ENUM_SILENTCHRGSTA_COMPLETE parameter; ENUM_SILENTCHRGSTA_FAULT parameter; ENUM_SILENTCHRGSTA_NONE parameter; FALSE parameter; TRUE parameter; VPMM_DCDCSetVCompleted_flg local boolean; VPMM_PrePwrSta_enum local double; KPMM_OFFStaByPassLVBatt_flg input; VINP_OBCPluginSta_flg input; VPMM_ChrgPlugFallingEdge_flg input; VPMM_SeatSWRisingEdge_flg input; VPMM_LVBattChrgtime_s local double; ENUM_SILENTCHRGLV_LV3 parameter; VINP_SchedChgbutt_flg input; VPMM_MCUDCBusMaxVolt_V input; VINP_DrDoorSW_flg input; VPMM_LVBattChktime_s output; KPMM_MCUDischrgVolt_V parameter; KPMM_PwrStaOFFCTO_s parameter; KPMM_PwrStaONTO_s parameter; VINP_HoodSW_flg input; VINP_AllowMovThd_OTA_enum input; VPMM_PwrStaOFFCTimer_s local single; VPMM_PwrStaONTimer_s local double; ENUM_ALLOWMOV_ALLOWREADY parameter; ENUM_PWRCONSTRAINT_ONFORTIME parameter; ENUM_PWRCONSTRAINT_PWRSTAON parameter; ENUM_PWRDOWNREQ_SYSREQPD parameter; ENUM_PWRDOWNREQ_USERREQPD parameter; ENUM_PWRSTASELECT_GOOFFA parameter; ENUM_PWRSTASELECT_GOOFFC parameter; ENUM_PWRSTASELECT_GOON parameter; ENUM_PWRSTATOSTA_NORMAL parameter; ENUM_PWRSTATOSTA_TIMEOUT parameter; ENUM_PWRUPREQ_SYSREQPU parameter; ENUM_PWRUPREQ_USERREQPU parameter; KPMM_Sched_ChgTO_s parameter; VPMM_SchedChgTOTimer_s local single; ENUM_SCHEDCHGTO_NORMAL parameter; ENUM_SCHEDCHGTO_TIMEOUT parameter; VPMM_LVSilentChrgReq_flg output; VPMM_PwrStaTOSta_enum output; VPMM_PwrDownReq_enum input; VPMM_PwrStaConstraint_enum input; VPMM_PwrStaSelect_enum input; VPMM_PwrUpReq_enum input; VINP_CANMsgValidBMS3_flg input; KPMM_CANValidChkFailtime_s parameter; VPMM_CANMsgValid_flg local boolean; VPMM_CANValidChkFailtimer_s local single; VPMM_FirstEnterOFF_flg local boolean; VPMM_Sched_ChgTOSta_enum output; VINP_PwrReq_OTA_enum input; VDHP_ActAPSPosn_pct input; KPMM_LVBattChkOKStdT_s input; KPMM_PwrStaStdTO_s input; VPMM_LVSilentChrgReqStd_flg output; VPMM_LVBattChkOKStdTtimer_s local single; VPMM_PwrStaStdTOtimer_s local single; ENUM_PWRREQOTA_REQPOWERSTDBY parameter; VDHP_EAPS12RangeSta_enum input; VPMM_IVIPwrOffMemory_flg local boolean; VPMM_PreOFF_flg output; VINP_VehSpeed_kph input; KPMM_APSAllowThd_pct input; KPMM_PluginVehSpdThd_kph input; KPMM_LVChrgCurrMthd_flg input; KPMM_LVChrgHoldT_s input; KPMM_SysBaseCurr_A input; VINP_CoolgFanActDuty_pct input; VINP_DCDCAuxCur_A input; VINP_FDEWP1Cmd_enum input; VINP_FDEWP3Cmd_enum input; VPMM_CoolgFanActCurr_A local single; VPMM_EWP1Curr_A local single; VPMM_EWP3Curr_A local single; VPMM_LVChrgCurrThd_A local single; VPMM_LVSilentChrgSta_enum output; VPMM_DetectPDKeyUnlock_flg input; VPMM_DetectAntitheftLock_flg input; VPMM_DetectPDKeyLock_flg input; VPMM_DetectIVIPwroffreq_flg input; VPMM_DetectSchedChg_flg input; VPMM_DetectPWCONTINUE_flg input; VPMM_ContinueUseHold_flg local boolean; VPMM_PwrStaONTOPopT_s local single; VPMM_PwrStaONTOPop_s local single; ENUM_CHRGPLUGSTA_AC parameter; VPMM_PwrStaONTOPopReq_flg output; VPMM_IVIPwrStaONTOPopT_s output; VPMM_LVChrgHoldTtimer_s output; VPMM_LVBattChrgTimeCnt_s output; KPMM_SilentChrgReqTO_s input; VPMM_SilentChrgReqTimer_s local single; KPMM_PwrStaONTOPop_s input; KPMM_FDADC12VDetAccuIntval_s input; KPMM_FDADC12VDetAccu_s input; KPMM_FirstLVCheckHoldT_s input; KPMM_LVBattChkWakehold_s input; KPMM_LVBattOFFSlpThd_mV input; KPMM_OFFLVBattChkRetry_cnt input; VINP_LvBattVolt_mV input; VPMM_PMMAllowECUSleep_flg output; VPMM_FDADC12VDetAccuTimer_s local double; VPMM_FDADC12VDetAccu_cnt local double; VPMM_FDADC12VDetbuff_mV local single; VPMM_FirstFDADC12VDetAvg_mV local single; VPMM_FirstLVCheckHoldTimer_s local double; VPMM_LVBatStaChk_flg local boolean; VPMM_LVBattChkWakeholdTimer_s local single; VPMM_OFFLVBattChkRechkDone_flg local boolean; VPMM_OFFLVBattChkRechk_cnt local double; VPMM_SilentChkAllowSleep_flg output; VPMM_TimerAllowSleep_flg output; VPMM_FDADC12VDetAvg_mV output single; VPMM_LVSilentChrgLv_enum output; VINP_CANMsgValidBMS5_flg input; KPMM_BattUpResetRty_cnt input; KPMM_BattUpResetSW_flg input; KPMM_BattUpResetTO_s input; KPMM_BattUpRstDlyTO_s input; VINP_BMSWarn6_flg input; VINP_TailgateSW_flg input; VPMM_CtrlDrPwrStbA2_flg output; VPMM_CtrlFrBMSCCUCIR_flg output; VPMM_CtrlFrEDUINVERTER_flg output; VPMM_CtrlFrPwrStbA1P_flg output; VPMM_CtrlFrRC1_flg output; VPMM_HWResetSta_enum output; VPMM_BattUpResetRty_cnt local uint8; VPMM_BattUpResetTO_s local single; VPMM_BattUpReset_flg local boolean; VPMM_BattUpRstDlyTO_s local single; VPMM_HardwareRst_flg local boolean; ENUM_RANGESTA_12OUT parameter; VPMM_HVChrgPreActionErrSta_enum output double; KPMM_HoodOffChkFailtime_s input; VPMM_HoodOffChkFailtimer_s local single; VPMM_HoodOffStaChk_flg local boolean; KPMM_HVSOCWarnThd_pct input; VINP_OFFACMODE_enum input; VINP_V2LSta_enum input; ENUM_V2LSTA_NOPLUG parameter; VINP_PsDoorSW_flg input; VINP_RRDoorSW_flg input; VINP_RLDoorSW_flg input; VPMM_DetectPsDoorOpened_flg input; VPMM_DetectRLDoorOpened_flg input; VPMM_DetectRRDoorOpened_flg input; VPMM_DetectSeatEmpty_flg input; ENUM_OFFACMODE_INVALID parameter; ENUM_OFFACMODE_OFF parameter; VPMM_PMMAllowNMSleep_flg output boolean; VPMM_SilentChrgFaultBypass_flg local double; ENUM_PWRREQOTA_REQPOWERON parameter; VPMM_FDADC12VDetAvgTMP_mV local single; VPMM_PCUPwrUpDelayDone_flg local boolean; VPMM_TimePCUDelay_s local single; KPMM_PCUPwrUpDelayTime_s parameter; VPMM_PDUDCDCRlyDone_flg local boolean; KPMM_PCUDCDCRlyEnByPassSW_flg parameter; KPMM_PCUChkFailTime_s parameter; KPMM_PCUEACRlyEnByPassSW_flg parameter; VINP_PDUDCDCRlySta_enum input; VINP_PDUEACRlySta_enum input; VPMM_DCDCRlyDem_enum output; VPMM_EACRlyDem_enum output; ENUM_PCUPUSTA_DCDCRELAYFAIL parameter; ENUM_PCUPUSTA_NORMAL parameter; VPMM_TimePDUEACRlyEnable_s local single; VPMM_TimePDUDCDCRlyEnable_s local single; VPMM_PDUEACRlyDone_flg local boolean; VPMM_TimePDUEHPSRlyEnable_s local single; KPMM_PCUEHPSRlyEnByPassSW_flg parameter; VINP_DCDCEnSta_enum input; VINP_PDUEHPSRlySta_enum input; VPMM_DCDCEnDem_enum output; ENUM_DCDCENSTA_RUN parameter; ENUM_DCDCENDEM_START parameter; VPMM_PDUDCDCEnableDone_flg local boolean; VPMM_PDUEHPSRlyDone_flg local boolean; VPMM_PCUPwrUpFaultSta_enum local uint8; VPMM_EHPSRlyDem_enum output; VPMM_TimePDUDCDCEnable_s local single; ENUM_PCUPUSTA_24VDCDCENABLEFAIL parameter; ENUM_PCUPUSTA_EACRELAYFAIL parameter; ENUM_PCUPUSTA_EHPSRELAYFAIL parameter; ENUM_DCDCRLYDEM_ENABLE parameter; ENUM_EACRLYDEM_ENABLE parameter; ENUM_EHPSRLYDEM_ENABLE parameter; ENUM_PDUDCDCRLYSTA_CLOSE parameter; ENUM_PDUEACRLYSTA_CLOSE parameter; ENUM_PDUEHPSRLYSTA_CLOSE parameter; ENUM_DCDCENSTA_READY parameter; ENUM_DCDCENDEM_SHUTDOWN parameter; VINP_EACEnSta_enum input; VINP_EHPSEnSta_enum input; ENUM_PCUPDSTA_PCUDISABLEFAIL parameter; VPMM_PCUDCDCPD1Completed_flg local boolean; VPMM_TimePCUDCDCDisable_s local single; ENUM_EACENSTA_READY parameter; ENUM_EHPSENSTA_READY parameter; ENUM_PDUDCDCRLYSTA_OPEN parameter; ENUM_PDUEACRLYSTA_OPEN parameter; ENUM_PDUEHPSRLYSTA_OPEN parameter; ENUM_EHPSRLYDEM_DISABLE parameter; ENUM_EACRLYDEM_DISABLE parameter; ENUM_DCDCRLYDEM_DISABLE parameter; VPMM_PCUDCDCPD2Completed_flg local boolean; VPMM_OFFPBRisingEdge_flg input; VPMM_STBPBRisingEdge_flg input; VPMM_ONPBRisingEdge_flg input; VPMM_ONPBSta_flg input; VPMM_READYPBRisingEdge_flg input; VPMM_OFFAPBRisingEdge_flg input; VPMM_OFFCPBRisingEdge_flg input; VPMM_LVSilentChrgLv12V_enum local uint8; VPMM_SilentChkAllowSleep12V_flg local boolean; VPMM_LVSilentChrgReq12V_flg local boolean; VPMM_PMMAllowNMSleep12V_flg local boolean; VINP_LvBattVolt24V_mV input; KPMM_LVBattOFFSlpThd24V_mV input; KPMM_FDADC24VDetAccuIntval_s input; VPMM_FDADC24VDetAccu_cnt local double; VPMM_FDADC24VDetAccuTimer_s local double; VPMM_LVSilentChrgLv24V_enum local uint8; VPMM_SilentChkAllowSleep24V_flg local boolean; VPMM_PMMAllowNMSleep24V_flg local boolean; VPMM_FDADC24VDetAvg_mV local single; KPMM_FDADC24VDetAccu_s input; VPMM_LVSilentChrgReq24V_flg local boolean; VPMM_FirstFDADC24VDetAvg_mV local single; VPMM_FDADC24VDetAvgTMP_mV local single; VPMM_FDADC24VDetbuff_mV local single; VINP_CANMsgValidDCDCStatus2_flg input; KPMM_LVBattThd24V_V input; VINP_LVBattDet24V_V input; VINP_FDDoorstate_enum input; ENUM_FDDOORSTA_OPEN parameter; VPMM_READYPBMemory_flg input; VPMM_UserLeaveTChk_flg input; VINP_FDDoorOpen_enum input; VACC_EACPreSelfChkSta_flg input; VPMM_PwrUpPBPress_flg input; ENUM_POWERSTA_PWRUP parameter; ENUM_POWERSTA_PWRDOWN parameter; VPMM_24VCANMsgValid_flg local boolean; VPMM_24VCANValidChkFailtimer_s local single; VPMM_24VFirstLVCheckHoldTimer_s local single; VPMM_24VLVBatStaChk_flg local boolean; VPMM_24VOFFLVBattChkRechkDone_flg local boolean; VPMM_24VOFFLVBattChkRechk_cnt local single; ENUM_PCUPDSTA_NORMAL parameter; ENUM_PCUPDSTA_PCURELAYOPENFAIL parameter; VPMM_PCUPwrDowFaultSta_enum local uint8
